simulink model "OverlapSaveFIR_11paths"  (R2024a)
settings: Solver=VariableStepAuto  StartTime=0.0  StopTime=8192  RelTol=1e-3
InitFcn:
  | N=256;
  | h=firpm(128,[0;0.4;0.5;1],[1;1;0;0],[1;50],{20});
  | hc=fft(h,N);
  | h_quant = int16(2^14*hc/max(hc));
  | M=length(h);
values from neighbouring files (symbols this model uses):
  tmp = double(int16(tmp*2^16))/2^16    [test_tap32_fft128.m]
undefined symbols (not defined in the file or in its folder): S, vsva2197, xcvc1902
libraries: aieBasic x44, aieUtilities x11, dspxfrm3 x2, dspsrcs4 x2, vmcUtilities x1
(part 2 of 2)

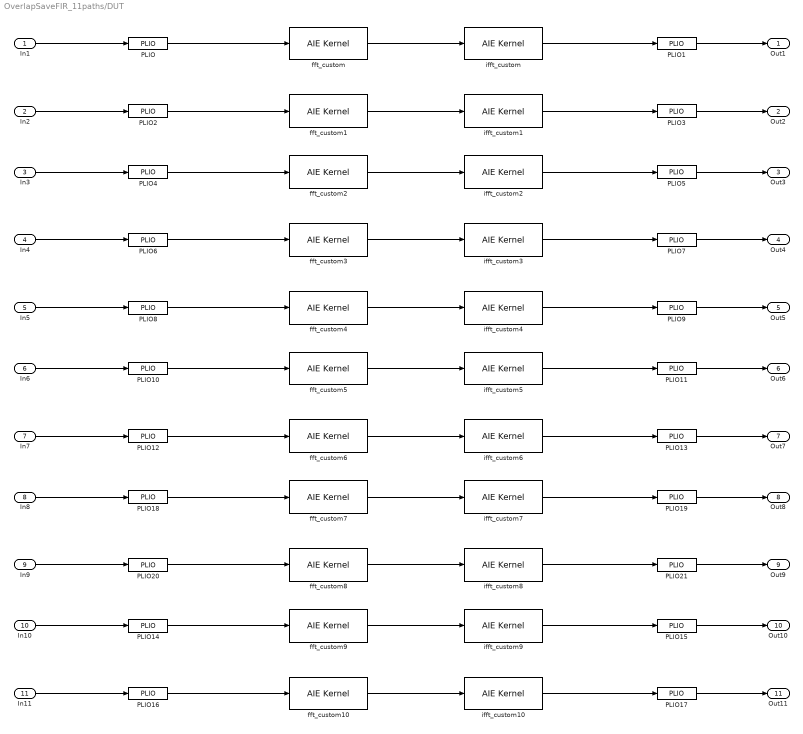
== system OverlapSaveFIR_11paths/DUT ==
  In1 : Inport
  In2 : Inport  Port=2
  In3 : Inport  Port=3
  In4 : Inport  Port=4
  In5 : Inport  Port=5
  In6 : Inport  Port=6
  In7 : Inport  Port=7
  In8 : Inport  Port=8
  In9 : Inport  Port=9
  In10 : Inport  Port=10
  In11 : Inport  Port=11
  PLIO{,1..21} (22 alike) : aieBasic/PLIO  PlioWidth=64  PlioFreqSpec=on  PlioFreq=625  ColLocation=0  channel=0  blockJsonConstraints=[]  deprecateConstraints=0
  fft_custom : aieBasic/AIE Kernel  KernelAllAttrs=s[12;12;9;9;19;14;21;23;21;23;24;21;15;17;12;24;26;26;26;27;28;9;21;23;23;23;24;25;14;19;19;29]@FunctionNameDeclFileNamePortNamesPortTypesPortSerializedTypesPortDirectionsPortWindowSizeEnablesPortWindowMarginEnablesPortBufferSizeEnablesPortBufferMarginEnablesPortSynchronicityEnablesPortSignalSizeEnablesPortBufferSizesPortBufferMarginsFunctionDeclFunctionTemplateSpecKindFunctionTemplateParamNamesFunctionTemplateParamKindsFunctionTemplateParamTypesFunctionTemplateParamValuesFunctionTemplateParamEnablesClassDeclClassTemplateSpecKindClassTemplateParamNamesClassTemplateParamKindsClassTemplateParamTypesClassTemplateParamValuesClassTemplateParamEnablesClassCtorDeclsClassCtorParamNamesClassCtorParamTypesClassCtorParamSerializedTypes[1 1]@C[32 1]@t10@fft_customt33@../../customFFT_casc/fft_custom.hC[2 1]@t5@sig_it5@sig_oC[2 1]@t59@adf::input_buffer< cint32, adf::extents< 256 > > & restrictt32@output_cascade< cacc48, void > *C[2 1]@t71@{Q2{R{Tadf::input_buffer{2{t{Scint32}}{t{Tadf::extents{1{t{}256}}}}}}}}t42@{P{Toutput_cascade{2{t{Scacc48}}{t{Bv}}}}}C[2 1]@t5@inputt6@outputC[2 1]@l1@l0@C[2 1]@l1@l0@C[2 1]@l1@l0@C[2 1]@l0@l0@C[2 1]@l1@l0@C[2 1]@l0@l1@C[2 1]@t3@256nC[2 1]@nnt122@void fft_custom(adf::input_buffer< cint32, adf::extents< 256 > > & restrict sig_i, output_cascade< cacc48, void > * sig_o)t4@nonee[0 1]@e[0 1]@e[0 1]@e[0 1]@e[0 1]@nne[0 1]@e[0 1]@e[0 1]@e[0 1]@e[0 1]@e[0 1]@e[0 1]@e[0 1]@e[0 1]@  PortNames={'sig_i'; 'sig_o'}  PortSerializedTypes={'{Q2{R{Tadf::input_buffer{2{t{Scint32}}{t{Tadf::extents{1{t{}256}}}}}}}}'; '{P{Toutput_cascade{2{t{Scacc48}}{t{Bv}}}}}'}  PortWindowSizes={2.560000000000000000e+02, 0.000000000000000000e+00}  PortWindowMargins={0.000000000000000000e+00, 0.000000000000000000e+00}  PortSynchronicities={'sync', 'auto'}  PortSignalSizes={0.000000000000000000e+00; 2.560000000000000000e+02}  FunctionTemplateSpecKind=none  FunctionTemplateParamNames={}  FunctionTemplateParamKinds={}  FunctionTemplateParamTypes={}  FunctionTemplateParamValues={}  FunctionIndex=1  FunctionTabVisible=on  FunctionTemplateParamsVisible=off  FunctionDeclTypeOptions=C[1 1]@t123@void fft_custom(adf::input_buffer< cint32, adf::extents< 256 > > && restrict sig_i, output_cascade< cacc48, void > * sig_o)  FunctionDecl=void fft_custom(adf::input_buffer< cint32, adf::extents< 256 > > && restrict sig_i, output_cascade< cacc48, void > * sig_o)  FunctionTemplateParams={}  FunctionTemplateParamsEnables={}  PortAttrs={ 'input', 'sig_i', 'adf::input_buffer< cint32, adf::extents< 256 > > & restrict', '256', '0', 'sync', ''; 'output', 'sig_o', 'output_cascade< cacc48, void > *', '', '', '', '256' }  PortAttrsEnables={'off', 'off', 'off', 'off', 'off', 'off', 'off';'off', 'off', 'off', 'off', 'off', 'off', 'on'}  SampleTime=-1  KernelHeaderFile=customFFT_casc/fft_custom.h  KernelFunction=fft_custom  KernelInitFunction=fft_custom_init  KernelSourceFile=customFFT_casc/fft_custom.cpp  KernelSearchPaths={'./customFFT_casc'}  PreProcOptions={}  blockJsonConstraints="{\"type\":\"constraint\",\"constraintType\":\"stackSize\",\"sid\":\"5803\",\"lhs\":{\"type\":\"stackSize\",\"args\":{\"type\":\"kernel\",\"name\":\"OverlapSaveFIR_11paths/custom_11copies/fft_custom\",\"sid\":\"5803\"}},\"rhs\":{\"type\":\"value\",\"args\":{\"type\":\"evaluable\",\"expr\":\"3200\",\"value\":3200}},\"equality\":true}"
  fft_custom1 : aieBasic/AIE Kernel  KernelAllAttrs=s[12;12;9;9;19;14;21;23;21;23;24;21;15;17;12;24;26;26;26;27;28;9;21;23;23;23;24;25;14;19;19;29]@FunctionNameDeclFileNamePortNamesPortTypesPortSerializedTypesPortDirectionsPortWindowSizeEnablesPortWindowMarginEnablesPortBufferSizeEnablesPortBufferMarginEnablesPortSynchronicityEnablesPortSignalSizeEnablesPortBufferSizesPortBufferMarginsFunctionDeclFunctionTemplateSpecKindFunctionTemplateParamNamesFunctionTemplateParamKindsFunctionTemplateParamTypesFunctionTemplateParamValuesFunctionTemplateParamEnablesClassDeclClassTemplateSpecKindClassTemplateParamNamesClassTemplateParamKindsClassTemplateParamTypesClassTemplateParamValuesClassTemplateParamEnablesClassCtorDeclsClassCtorParamNamesClassCtorParamTypesClassCtorParamSerializedTypes[1 1]@C[32 1]@t10@fft_customt33@../../customFFT_casc/fft_custom.hC[2 1]@t5@sig_it5@sig_oC[2 1]@t59@adf::input_buffer< cint32, adf::extents< 256 > > & restrictt32@output_cascade< cacc48, void > *C[2 1]@t71@{Q2{R{Tadf::input_buffer{2{t{Scint32}}{t{Tadf::extents{1{t{}256}}}}}}}}t42@{P{Toutput_cascade{2{t{Scacc48}}{t{Bv}}}}}C[2 1]@t5@inputt6@outputC[2 1]@l1@l0@C[2 1]@l1@l0@C[2 1]@l1@l0@C[2 1]@l0@l0@C[2 1]@l1@l0@C[2 1]@l0@l1@C[2 1]@t3@256nC[2 1]@nnt122@void fft_custom(adf::input_buffer< cint32, adf::extents< 256 > > & restrict sig_i, output_cascade< cacc48, void > * sig_o)t4@nonee[0 1]@e[0 1]@e[0 1]@e[0 1]@e[0 1]@nne[0 1]@e[0 1]@e[0 1]@e[0 1]@e[0 1]@e[0 1]@e[0 1]@e[0 1]@e[0 1]@  PortNames={'sig_i'; 'sig_o'}  PortSerializedTypes={'{Q2{R{Tadf::input_buffer{2{t{Scint32}}{t{Tadf::extents{1{t{}256}}}}}}}}'; '{P{Toutput_cascade{2{t{Scacc48}}{t{Bv}}}}}'}  PortWindowSizes={2.560000000000000000e+02, 0.000000000000000000e+00}  PortWindowMargins={0.000000000000000000e+00, 0.000000000000000000e+00}  PortSynchronicities={'sync', 'auto'}  PortSignalSizes={0.000000000000000000e+00; 2.560000000000000000e+02}  FunctionTemplateSpecKind=none  FunctionTemplateParamNames={}  FunctionTemplateParamKinds={}  FunctionTemplateParamTypes={}  FunctionTemplateParamValues={}  FunctionIndex=1  FunctionTabVisible=on  FunctionTemplateParamsVisible=off  FunctionDeclTypeOptions=C[1 1]@t123@void fft_custom(adf::input_buffer< cint32, adf::extents< 256 > > && restrict sig_i, output_cascade< cacc48, void > * sig_o)  FunctionDecl=void fft_custom(adf::input_buffer< cint32, adf::extents< 256 > > && restrict sig_i, output_cascade< cacc48, void > * sig_o)  FunctionTemplateParams={}  FunctionTemplateParamsEnables={}  PortAttrs={ 'input', 'sig_i', 'adf::input_buffer< cint32, adf::extents< 256 > > & restrict', '256', '0', 'sync', ''; 'output', 'sig_o', 'output_cascade< cacc48, void > *', '', '', '', '256' }  PortAttrsEnables={'off', 'off', 'off', 'off', 'off', 'off', 'off';'off', 'off', 'off', 'off', 'off', 'off', 'on'}  SampleTime=-1  KernelHeaderFile=customFFT_casc/fft_custom.h  KernelFunction=fft_custom  KernelInitFunction=fft_custom_init  KernelSourceFile=customFFT_casc/fft_custom.cpp  KernelSearchPaths={'./customFFT_casc'}  PreProcOptions={}  blockJsonConstraints="{\"type\":\"constraint\",\"constraintType\":\"stackSize\",\"sid\":\"5804\",\"lhs\":{\"type\":\"stackSize\",\"args\":{\"type\":\"kernel\",\"name\":\"OverlapSaveFIR_11paths/custom_11copies/fft_custom1\",\"sid\":\"5804\"}},\"rhs\":{\"type\":\"value\",\"args\":{\"type\":\"evaluable\",\"expr\":\"3200\",\"value\":3200}},\"equality\":true}"
  fft_custom10 : aieBasic/AIE Kernel  KernelAllAttrs=s[12;12;9;9;19;14;21;23;21;23;24;21;15;17;12;24;26;26;26;27;28;9;21;23;23;23;24;25;14;19;19;29]@FunctionNameDeclFileNamePortNamesPortTypesPortSerializedTypesPortDirectionsPortWindowSizeEnablesPortWindowMarginEnablesPortBufferSizeEnablesPortBufferMarginEnablesPortSynchronicityEnablesPortSignalSizeEnablesPortBufferSizesPortBufferMarginsFunctionDeclFunctionTemplateSpecKindFunctionTemplateParamNamesFunctionTemplateParamKindsFunctionTemplateParamTypesFunctionTemplateParamValuesFunctionTemplateParamEnablesClassDeclClassTemplateSpecKindClassTemplateParamNamesClassTemplateParamKindsClassTemplateParamTypesClassTemplateParamValuesClassTemplateParamEnablesClassCtorDeclsClassCtorParamNamesClassCtorParamTypesClassCtorParamSerializedTypes[1 1]@C[32 1]@t10@fft_customt33@../../customFFT_casc/fft_custom.hC[2 1]@t5@sig_it5@sig_oC[2 1]@t59@adf::input_buffer< cint32, adf::extents< 256 > > & restrictt32@output_cascade< cacc48, void > *C[2 1]@t71@{Q2{R{Tadf::input_buffer{2{t{Scint32}}{t{Tadf::extents{1{t{}256}}}}}}}}t42@{P{Toutput_cascade{2{t{Scacc48}}{t{Bv}}}}}C[2 1]@t5@inputt6@outputC[2 1]@l1@l0@C[2 1]@l1@l0@C[2 1]@l1@l0@C[2 1]@l0@l0@C[2 1]@l1@l0@C[2 1]@l0@l1@C[2 1]@t3@256nC[2 1]@nnt122@void fft_custom(adf::input_buffer< cint32, adf::extents< 256 > > & restrict sig_i, output_cascade< cacc48, void > * sig_o)t4@nonee[0 1]@e[0 1]@e[0 1]@e[0 1]@e[0 1]@nne[0 1]@e[0 1]@e[0 1]@e[0 1]@e[0 1]@e[0 1]@e[0 1]@e[0 1]@e[0 1]@  PortNames={'sig_i'; 'sig_o'}  PortSerializedTypes={'{Q2{R{Tadf::input_buffer{2{t{Scint32}}{t{Tadf::extents{1{t{}256}}}}}}}}'; '{P{Toutput_cascade{2{t{Scacc48}}{t{Bv}}}}}'}  PortWindowSizes={2.560000000000000000e+02, 0.000000000000000000e+00}  PortWindowMargins={0.000000000000000000e+00, 0.000000000000000000e+00}  PortSynchronicities={'sync', 'auto'}  PortSignalSizes={0.000000000000000000e+00; 2.560000000000000000e+02}  FunctionTemplateSpecKind=none  FunctionTemplateParamNames={}  FunctionTemplateParamKinds={}  FunctionTemplateParamTypes={}  FunctionTemplateParamValues={}  FunctionIndex=1  FunctionTabVisible=on  FunctionTemplateParamsVisible=off  FunctionDeclTypeOptions=C[1 1]@t123@void fft_custom(adf::input_buffer< cint32, adf::extents< 256 > > && restrict sig_i, output_cascade< cacc48, void > * sig_o)  FunctionDecl=void fft_custom(adf::input_buffer< cint32, adf::extents< 256 > > && restrict sig_i, output_cascade< cacc48, void > * sig_o)  FunctionTemplateParams={}  FunctionTemplateParamsEnables={}  PortAttrs={ 'input', 'sig_i', 'adf::input_buffer< cint32, adf::extents< 256 > > & restrict', '256', '0', 'sync', ''; 'output', 'sig_o', 'output_cascade< cacc48, void > *', '', '', '', '256' }  PortAttrsEnables={'off', 'off', 'off', 'off', 'off', 'off', 'off';'off', 'off', 'off', 'off', 'off', 'off', 'on'}  SampleTime=-1  KernelHeaderFile=customFFT_casc/fft_custom.h  KernelFunction=fft_custom  KernelInitFunction=fft_custom_init  KernelSourceFile=customFFT_casc/fft_custom.cpp  KernelSearchPaths={'./customFFT_casc'}  PreProcOptions={}  blockJsonConstraints="{\"type\":\"constraint\",\"constraintType\":\"stackSize\",\"sid\":\"5805\",\"lhs\":{\"type\":\"stackSize\",\"args\":{\"type\":\"kernel\",\"name\":\"OverlapSaveFIR_11paths/custom_11copies/fft_custom10\",\"sid\":\"5805\"}},\"rhs\":{\"type\":\"value\",\"args\":{\"type\":\"evaluable\",\"expr\":\"3200\",\"value\":3200}},\"equality\":true}"
  fft_custom2 : aieBasic/AIE Kernel  KernelAllAttrs=s[12;12;9;9;19;14;21;23;21;23;24;21;15;17;12;24;26;26;26;27;28;9;21;23;23;23;24;25;14;19;19;29]@FunctionNameDeclFileNamePortNamesPortTypesPortSerializedTypesPortDirectionsPortWindowSizeEnablesPortWindowMarginEnablesPortBufferSizeEnablesPortBufferMarginEnablesPortSynchronicityEnablesPortSignalSizeEnablesPortBufferSizesPortBufferMarginsFunctionDeclFunctionTemplateSpecKindFunctionTemplateParamNamesFunctionTemplateParamKindsFunctionTemplateParamTypesFunctionTemplateParamValuesFunctionTemplateParamEnablesClassDeclClassTemplateSpecKindClassTemplateParamNamesClassTemplateParamKindsClassTemplateParamTypesClassTemplateParamValuesClassTemplateParamEnablesClassCtorDeclsClassCtorParamNamesClassCtorParamTypesClassCtorParamSerializedTypes[1 1]@C[32 1]@t10@fft_customt33@../../customFFT_casc/fft_custom.hC[2 1]@t5@sig_it5@sig_oC[2 1]@t59@adf::input_buffer< cint32, adf::extents< 256 > > & restrictt32@output_cascade< cacc48, void > *C[2 1]@t71@{Q2{R{Tadf::input_buffer{2{t{Scint32}}{t{Tadf::extents{1{t{}256}}}}}}}}t42@{P{Toutput_cascade{2{t{Scacc48}}{t{Bv}}}}}C[2 1]@t5@inputt6@outputC[2 1]@l1@l0@C[2 1]@l1@l0@C[2 1]@l1@l0@C[2 1]@l0@l0@C[2 1]@l1@l0@C[2 1]@l0@l1@C[2 1]@t3@256nC[2 1]@nnt122@void fft_custom(adf::input_buffer< cint32, adf::extents< 256 > > & restrict sig_i, output_cascade< cacc48, void > * sig_o)t4@nonee[0 1]@e[0 1]@e[0 1]@e[0 1]@e[0 1]@nne[0 1]@e[0 1]@e[0 1]@e[0 1]@e[0 1]@e[0 1]@e[0 1]@e[0 1]@e[0 1]@  PortNames={'sig_i'; 'sig_o'}  PortSerializedTypes={'{Q2{R{Tadf::input_buffer{2{t{Scint32}}{t{Tadf::extents{1{t{}256}}}}}}}}'; '{P{Toutput_cascade{2{t{Scacc48}}{t{Bv}}}}}'}  PortWindowSizes={2.560000000000000000e+02, 0.000000000000000000e+00}  PortWindowMargins={0.000000000000000000e+00, 0.000000000000000000e+00}  PortSynchronicities={'sync', 'auto'}  PortSignalSizes={0.000000000000000000e+00; 2.560000000000000000e+02}  FunctionTemplateSpecKind=none  FunctionTemplateParamNames={}  FunctionTemplateParamKinds={}  FunctionTemplateParamTypes={}  FunctionTemplateParamValues={}  FunctionIndex=1  FunctionTabVisible=on  FunctionTemplateParamsVisible=off  FunctionDeclTypeOptions=C[1 1]@t123@void fft_custom(adf::input_buffer< cint32, adf::extents< 256 > > && restrict sig_i, output_cascade< cacc48, void > * sig_o)  FunctionDecl=void fft_custom(adf::input_buffer< cint32, adf::extents< 256 > > && restrict sig_i, output_cascade< cacc48, void > * sig_o)  FunctionTemplateParams={}  FunctionTemplateParamsEnables={}  PortAttrs={ 'input', 'sig_i', 'adf::input_buffer< cint32, adf::extents< 256 > > & restrict', '256', '0', 'sync', ''; 'output', 'sig_o', 'output_cascade< cacc48, void > *', '', '', '', '256' }  PortAttrsEnables={'off', 'off', 'off', 'off', 'off', 'off', 'off';'off', 'off', 'off', 'off', 'off', 'off', 'on'}  SampleTime=-1  KernelHeaderFile=customFFT_casc/fft_custom.h  KernelFunction=fft_custom  KernelInitFunction=fft_custom_init  KernelSourceFile=customFFT_casc/fft_custom.cpp  KernelSearchPaths={'./customFFT_casc'}  PreProcOptions={}  blockJsonConstraints="{\"type\":\"constraint\",\"constraintType\":\"stackSize\",\"sid\":\"5806\",\"lhs\":{\"type\":\"stackSize\",\"args\":{\"type\":\"kernel\",\"name\":\"OverlapSaveFIR_11paths/custom_11copies/fft_custom2\",\"sid\":\"5806\"}},\"rhs\":{\"type\":\"value\",\"args\":{\"type\":\"evaluable\",\"expr\":\"3200\",\"value\":3200}},\"equality\":true}"
  fft_custom3 : aieBasic/AIE Kernel  KernelAllAttrs=s[12;12;9;9;19;14;21;23;21;23;24;21;15;17;12;24;26;26;26;27;28;9;21;23;23;23;24;25;14;19;19;29]@FunctionNameDeclFileNamePortNamesPortTypesPortSerializedTypesPortDirectionsPortWindowSizeEnablesPortWindowMarginEnablesPortBufferSizeEnablesPortBufferMarginEnablesPortSynchronicityEnablesPortSignalSizeEnablesPortBufferSizesPortBufferMarginsFunctionDeclFunctionTemplateSpecKindFunctionTemplateParamNamesFunctionTemplateParamKindsFunctionTemplateParamTypesFunctionTemplateParamValuesFunctionTemplateParamEnablesClassDeclClassTemplateSpecKindClassTemplateParamNamesClassTemplateParamKindsClassTemplateParamTypesClassTemplateParamValuesClassTemplateParamEnablesClassCtorDeclsClassCtorParamNamesClassCtorParamTypesClassCtorParamSerializedTypes[1 1]@C[32 1]@t10@fft_customt33@../../customFFT_casc/fft_custom.hC[2 1]@t5@sig_it5@sig_oC[2 1]@t59@adf::input_buffer< cint32, adf::extents< 256 > > & restrictt32@output_cascade< cacc48, void > *C[2 1]@t71@{Q2{R{Tadf::input_buffer{2{t{Scint32}}{t{Tadf::extents{1{t{}256}}}}}}}}t42@{P{Toutput_cascade{2{t{Scacc48}}{t{Bv}}}}}C[2 1]@t5@inputt6@outputC[2 1]@l1@l0@C[2 1]@l1@l0@C[2 1]@l1@l0@C[2 1]@l0@l0@C[2 1]@l1@l0@C[2 1]@l0@l1@C[2 1]@t3@256nC[2 1]@nnt122@void fft_custom(adf::input_buffer< cint32, adf::extents< 256 > > & restrict sig_i, output_cascade< cacc48, void > * sig_o)t4@nonee[0 1]@e[0 1]@e[0 1]@e[0 1]@e[0 1]@nne[0 1]@e[0 1]@e[0 1]@e[0 1]@e[0 1]@e[0 1]@e[0 1]@e[0 1]@e[0 1]@  PortNames={'sig_i'; 'sig_o'}  PortSerializedTypes={'{Q2{R{Tadf::input_buffer{2{t{Scint32}}{t{Tadf::extents{1{t{}256}}}}}}}}'; '{P{Toutput_cascade{2{t{Scacc48}}{t{Bv}}}}}'}  PortWindowSizes={2.560000000000000000e+02, 0.000000000000000000e+00}  PortWindowMargins={0.000000000000000000e+00, 0.000000000000000000e+00}  PortSynchronicities={'sync', 'auto'}  PortSignalSizes={0.000000000000000000e+00; 2.560000000000000000e+02}  FunctionTemplateSpecKind=none  FunctionTemplateParamNames={}  FunctionTemplateParamKinds={}  FunctionTemplateParamTypes={}  FunctionTemplateParamValues={}  FunctionIndex=1  FunctionTabVisible=on  FunctionTemplateParamsVisible=off  FunctionDeclTypeOptions=C[1 1]@t123@void fft_custom(adf::input_buffer< cint32, adf::extents< 256 > > && restrict sig_i, output_cascade< cacc48, void > * sig_o)  FunctionDecl=void fft_custom(adf::input_buffer< cint32, adf::extents< 256 > > && restrict sig_i, output_cascade< cacc48, void > * sig_o)  FunctionTemplateParams={}  FunctionTemplateParamsEnables={}  PortAttrs={ 'input', 'sig_i', 'adf::input_buffer< cint32, adf::extents< 256 > > & restrict', '256', '0', 'sync', ''; 'output', 'sig_o', 'output_cascade< cacc48, void > *', '', '', '', '256' }  PortAttrsEnables={'off', 'off', 'off', 'off', 'off', 'off', 'off';'off', 'off', 'off', 'off', 'off', 'off', 'on'}  SampleTime=-1  KernelHeaderFile=customFFT_casc/fft_custom.h  KernelFunction=fft_custom  KernelInitFunction=fft_custom_init  KernelSourceFile=customFFT_casc/fft_custom.cpp  KernelSearchPaths={'./customFFT_casc'}  PreProcOptions={}  blockJsonConstraints="{\"type\":\"constraint\",\"constraintType\":\"stackSize\",\"sid\":\"5807\",\"lhs\":{\"type\":\"stackSize\",\"args\":{\"type\":\"kernel\",\"name\":\"OverlapSaveFIR_11paths/custom_11copies/fft_custom3\",\"sid\":\"5807\"}},\"rhs\":{\"type\":\"value\",\"args\":{\"type\":\"evaluable\",\"expr\":\"3200\",\"value\":3200}},\"equality\":true}"
  fft_custom4 : aieBasic/AIE Kernel  KernelAllAttrs=s[12;12;9;9;19;14;21;23;21;23;24;21;15;17;12;24;26;26;26;27;28;9;21;23;23;23;24;25;14;19;19;29]@FunctionNameDeclFileNamePortNamesPortTypesPortSerializedTypesPortDirectionsPortWindowSizeEnablesPortWindowMarginEnablesPortBufferSizeEnablesPortBufferMarginEnablesPortSynchronicityEnablesPortSignalSizeEnablesPortBufferSizesPortBufferMarginsFunctionDeclFunctionTemplateSpecKindFunctionTemplateParamNamesFunctionTemplateParamKindsFunctionTemplateParamTypesFunctionTemplateParamValuesFunctionTemplateParamEnablesClassDeclClassTemplateSpecKindClassTemplateParamNamesClassTemplateParamKindsClassTemplateParamTypesClassTemplateParamValuesClassTemplateParamEnablesClassCtorDeclsClassCtorParamNamesClassCtorParamTypesClassCtorParamSerializedTypes[1 1]@C[32 1]@t10@fft_customt33@../../customFFT_casc/fft_custom.hC[2 1]@t5@sig_it5@sig_oC[2 1]@t59@adf::input_buffer< cint32, adf::extents< 256 > > & restrictt32@output_cascade< cacc48, void > *C[2 1]@t71@{Q2{R{Tadf::input_buffer{2{t{Scint32}}{t{Tadf::extents{1{t{}256}}}}}}}}t42@{P{Toutput_cascade{2{t{Scacc48}}{t{Bv}}}}}C[2 1]@t5@inputt6@outputC[2 1]@l1@l0@C[2 1]@l1@l0@C[2 1]@l1@l0@C[2 1]@l0@l0@C[2 1]@l1@l0@C[2 1]@l0@l1@C[2 1]@t3@256nC[2 1]@nnt122@void fft_custom(adf::input_buffer< cint32, adf::extents< 256 > > & restrict sig_i, output_cascade< cacc48, void > * sig_o)t4@nonee[0 1]@e[0 1]@e[0 1]@e[0 1]@e[0 1]@nne[0 1]@e[0 1]@e[0 1]@e[0 1]@e[0 1]@e[0 1]@e[0 1]@e[0 1]@e[0 1]@  PortNames={'sig_i'; 'sig_o'}  PortSerializedTypes={'{Q2{R{Tadf::input_buffer{2{t{Scint32}}{t{Tadf::extents{1{t{}256}}}}}}}}'; '{P{Toutput_cascade{2{t{Scacc48}}{t{Bv}}}}}'}  PortWindowSizes={2.560000000000000000e+02, 0.000000000000000000e+00}  PortWindowMargins={0.000000000000000000e+00, 0.000000000000000000e+00}  PortSynchronicities={'sync', 'auto'}  PortSignalSizes={0.000000000000000000e+00; 2.560000000000000000e+02}  FunctionTemplateSpecKind=none  FunctionTemplateParamNames={}  FunctionTemplateParamKinds={}  FunctionTemplateParamTypes={}  FunctionTemplateParamValues={}  FunctionIndex=1  FunctionTabVisible=on  FunctionTemplateParamsVisible=off  FunctionDeclTypeOptions=C[1 1]@t123@void fft_custom(adf::input_buffer< cint32, adf::extents< 256 > > && restrict sig_i, output_cascade< cacc48, void > * sig_o)  FunctionDecl=void fft_custom(adf::input_buffer< cint32, adf::extents< 256 > > && restrict sig_i, output_cascade< cacc48, void > * sig_o)  FunctionTemplateParams={}  FunctionTemplateParamsEnables={}  PortAttrs={ 'input', 'sig_i', 'adf::input_buffer< cint32, adf::extents< 256 > > & restrict', '256', '0', 'sync', ''; 'output', 'sig_o', 'output_cascade< cacc48, void > *', '', '', '', '256' }  PortAttrsEnables={'off', 'off', 'off', 'off', 'off', 'off', 'off';'off', 'off', 'off', 'off', 'off', 'off', 'on'}  SampleTime=-1  KernelHeaderFile=customFFT_casc/fft_custom.h  KernelFunction=fft_custom  KernelInitFunction=fft_custom_init  KernelSourceFile=customFFT_casc/fft_custom.cpp  KernelSearchPaths={'./customFFT_casc'}  PreProcOptions={}  blockJsonConstraints="{\"type\":\"constraint\",\"constraintType\":\"stackSize\",\"sid\":\"5808\",\"lhs\":{\"type\":\"stackSize\",\"args\":{\"type\":\"kernel\",\"name\":\"OverlapSaveFIR_11paths/custom_11copies/fft_custom4\",\"sid\":\"5808\"}},\"rhs\":{\"type\":\"value\",\"args\":{\"type\":\"evaluable\",\"expr\":\"3200\",\"value\":3200}},\"equality\":true}"
  fft_custom5 : aieBasic/AIE Kernel  KernelAllAttrs=s[12;12;9;9;19;14;21;23;21;23;24;21;15;17;12;24;26;26;26;27;28;9;21;23;23;23;24;25;14;19;19;29]@FunctionNameDeclFileNamePortNamesPortTypesPortSerializedTypesPortDirectionsPortWindowSizeEnablesPortWindowMarginEnablesPortBufferSizeEnablesPortBufferMarginEnablesPortSynchronicityEnablesPortSignalSizeEnablesPortBufferSizesPortBufferMarginsFunctionDeclFunctionTemplateSpecKindFunctionTemplateParamNamesFunctionTemplateParamKindsFunctionTemplateParamTypesFunctionTemplateParamValuesFunctionTemplateParamEnablesClassDeclClassTemplateSpecKindClassTemplateParamNamesClassTemplateParamKindsClassTemplateParamTypesClassTemplateParamValuesClassTemplateParamEnablesClassCtorDeclsClassCtorParamNamesClassCtorParamTypesClassCtorParamSerializedTypes[1 1]@C[32 1]@t10@fft_customt33@../../customFFT_casc/fft_custom.hC[2 1]@t5@sig_it5@sig_oC[2 1]@t59@adf::input_buffer< cint32, adf::extents< 256 > > & restrictt32@output_cascade< cacc48, void > *C[2 1]@t71@{Q2{R{Tadf::input_buffer{2{t{Scint32}}{t{Tadf::extents{1{t{}256}}}}}}}}t42@{P{Toutput_cascade{2{t{Scacc48}}{t{Bv}}}}}C[2 1]@t5@inputt6@outputC[2 1]@l1@l0@C[2 1]@l1@l0@C[2 1]@l1@l0@C[2 1]@l0@l0@C[2 1]@l1@l0@C[2 1]@l0@l1@C[2 1]@t3@256nC[2 1]@nnt122@void fft_custom(adf::input_buffer< cint32, adf::extents< 256 > > & restrict sig_i, output_cascade< cacc48, void > * sig_o)t4@nonee[0 1]@e[0 1]@e[0 1]@e[0 1]@e[0 1]@nne[0 1]@e[0 1]@e[0 1]@e[0 1]@e[0 1]@e[0 1]@e[0 1]@e[0 1]@e[0 1]@  PortNames={'sig_i'; 'sig_o'}  PortSerializedTypes={'{Q2{R{Tadf::input_buffer{2{t{Scint32}}{t{Tadf::extents{1{t{}256}}}}}}}}'; '{P{Toutput_cascade{2{t{Scacc48}}{t{Bv}}}}}'}  PortWindowSizes={2.560000000000000000e+02, 0.000000000000000000e+00}  PortWindowMargins={0.000000000000000000e+00, 0.000000000000000000e+00}  PortSynchronicities={'sync', 'auto'}  PortSignalSizes={0.000000000000000000e+00; 2.560000000000000000e+02}  FunctionTemplateSpecKind=none  FunctionTemplateParamNames={}  FunctionTemplateParamKinds={}  FunctionTemplateParamTypes={}  FunctionTemplateParamValues={}  FunctionIndex=1  FunctionTabVisible=on  FunctionTemplateParamsVisible=off  FunctionDeclTypeOptions=C[1 1]@t123@void fft_custom(adf::input_buffer< cint32, adf::extents< 256 > > && restrict sig_i, output_cascade< cacc48, void > * sig_o)  FunctionDecl=void fft_custom(adf::input_buffer< cint32, adf::extents< 256 > > && restrict sig_i, output_cascade< cacc48, void > * sig_o)  FunctionTemplateParams={}  FunctionTemplateParamsEnables={}  PortAttrs={ 'input', 'sig_i', 'adf::input_buffer< cint32, adf::extents< 256 > > & restrict', '256', '0', 'sync', ''; 'output', 'sig_o', 'output_cascade< cacc48, void > *', '', '', '', '256' }  PortAttrsEnables={'off', 'off', 'off', 'off', 'off', 'off', 'off';'off', 'off', 'off', 'off', 'off', 'off', 'on'}  SampleTime=-1  KernelHeaderFile=customFFT_casc/fft_custom.h  KernelFunction=fft_custom  KernelInitFunction=fft_custom_init  KernelSourceFile=customFFT_casc/fft_custom.cpp  KernelSearchPaths={'./customFFT_casc'}  PreProcOptions={}  blockJsonConstraints="{\"type\":\"constraint\",\"constraintType\":\"stackSize\",\"sid\":\"5809\",\"lhs\":{\"type\":\"stackSize\",\"args\":{\"type\":\"kernel\",\"name\":\"OverlapSaveFIR_11paths/custom_11copies/fft_custom5\",\"sid\":\"5809\"}},\"rhs\":{\"type\":\"value\",\"args\":{\"type\":\"evaluable\",\"expr\":\"3200\",\"value\":3200}},\"equality\":true}"
  fft_custom6 : aieBasic/AIE Kernel  KernelAllAttrs=s[12;12;9;9;19;14;21;23;21;23;24;21;15;17;12;24;26;26;26;27;28;9;21;23;23;23;24;25;14;19;19;29]@FunctionNameDeclFileNamePortNamesPortTypesPortSerializedTypesPortDirectionsPortWindowSizeEnablesPortWindowMarginEnablesPortBufferSizeEnablesPortBufferMarginEnablesPortSynchronicityEnablesPortSignalSizeEnablesPortBufferSizesPortBufferMarginsFunctionDeclFunctionTemplateSpecKindFunctionTemplateParamNamesFunctionTemplateParamKindsFunctionTemplateParamTypesFunctionTemplateParamValuesFunctionTemplateParamEnablesClassDeclClassTemplateSpecKindClassTemplateParamNamesClassTemplateParamKindsClassTemplateParamTypesClassTemplateParamValuesClassTemplateParamEnablesClassCtorDeclsClassCtorParamNamesClassCtorParamTypesClassCtorParamSerializedTypes[1 1]@C[32 1]@t10@fft_customt33@../../customFFT_casc/fft_custom.hC[2 1]@t5@sig_it5@sig_oC[2 1]@t59@adf::input_buffer< cint32, adf::extents< 256 > > & restrictt32@output_cascade< cacc48, void > *C[2 1]@t71@{Q2{R{Tadf::input_buffer{2{t{Scint32}}{t{Tadf::extents{1{t{}256}}}}}}}}t42@{P{Toutput_cascade{2{t{Scacc48}}{t{Bv}}}}}C[2 1]@t5@inputt6@outputC[2 1]@l1@l0@C[2 1]@l1@l0@C[2 1]@l1@l0@C[2 1]@l0@l0@C[2 1]@l1@l0@C[2 1]@l0@l1@C[2 1]@t3@256nC[2 1]@nnt122@void fft_custom(adf::input_buffer< cint32, adf::extents< 256 > > & restrict sig_i, output_cascade< cacc48, void > * sig_o)t4@nonee[0 1]@e[0 1]@e[0 1]@e[0 1]@e[0 1]@nne[0 1]@e[0 1]@e[0 1]@e[0 1]@e[0 1]@e[0 1]@e[0 1]@e[0 1]@e[0 1]@  PortNames={'sig_i'; 'sig_o'}  PortSerializedTypes={'{Q2{R{Tadf::input_buffer{2{t{Scint32}}{t{Tadf::extents{1{t{}256}}}}}}}}'; '{P{Toutput_cascade{2{t{Scacc48}}{t{Bv}}}}}'}  PortWindowSizes={2.560000000000000000e+02, 0.000000000000000000e+00}  PortWindowMargins={0.000000000000000000e+00, 0.000000000000000000e+00}  PortSynchronicities={'sync', 'auto'}  PortSignalSizes={0.000000000000000000e+00; 2.560000000000000000e+02}  FunctionTemplateSpecKind=none  FunctionTemplateParamNames={}  FunctionTemplateParamKinds={}  FunctionTemplateParamTypes={}  FunctionTemplateParamValues={}  FunctionIndex=1  FunctionTabVisible=on  FunctionTemplateParamsVisible=off  FunctionDeclTypeOptions=C[1 1]@t123@void fft_custom(adf::input_buffer< cint32, adf::extents< 256 > > && restrict sig_i, output_cascade< cacc48, void > * sig_o)  FunctionDecl=void fft_custom(adf::input_buffer< cint32, adf::extents< 256 > > && restrict sig_i, output_cascade< cacc48, void > * sig_o)  FunctionTemplateParams={}  FunctionTemplateParamsEnables={}  PortAttrs={ 'input', 'sig_i', 'adf::input_buffer< cint32, adf::extents< 256 > > & restrict', '256', '0', 'sync', ''; 'output', 'sig_o', 'output_cascade< cacc48, void > *', '', '', '', '256' }  PortAttrsEnables={'off', 'off', 'off', 'off', 'off', 'off', 'off';'off', 'off', 'off', 'off', 'off', 'off', 'on'}  SampleTime=-1  KernelHeaderFile=customFFT_casc/fft_custom.h  KernelFunction=fft_custom  KernelInitFunction=fft_custom_init  KernelSourceFile=customFFT_casc/fft_custom.cpp  KernelSearchPaths={'./customFFT_casc'}  PreProcOptions={}  blockJsonConstraints="{\"type\":\"constraint\",\"constraintType\":\"stackSize\",\"sid\":\"5810\",\"lhs\":{\"type\":\"stackSize\",\"args\":{\"type\":\"kernel\",\"name\":\"OverlapSaveFIR_11paths/custom_11copies/fft_custom6\",\"sid\":\"5810\"}},\"rhs\":{\"type\":\"value\",\"args\":{\"type\":\"evaluable\",\"expr\":\"3200\",\"value\":3200}},\"equality\":true}"
  fft_custom7 : aieBasic/AIE Kernel  KernelAllAttrs=s[12;12;9;9;19;14;21;23;21;23;24;21;15;17;12;24;26;26;26;27;28;9;21;23;23;23;24;25;14;19;19;29]@FunctionNameDeclFileNamePortNamesPortTypesPortSerializedTypesPortDirectionsPortWindowSizeEnablesPortWindowMarginEnablesPortBufferSizeEnablesPortBufferMarginEnablesPortSynchronicityEnablesPortSignalSizeEnablesPortBufferSizesPortBufferMarginsFunctionDeclFunctionTemplateSpecKindFunctionTemplateParamNamesFunctionTemplateParamKindsFunctionTemplateParamTypesFunctionTemplateParamValuesFunctionTemplateParamEnablesClassDeclClassTemplateSpecKindClassTemplateParamNamesClassTemplateParamKindsClassTemplateParamTypesClassTemplateParamValuesClassTemplateParamEnablesClassCtorDeclsClassCtorParamNamesClassCtorParamTypesClassCtorParamSerializedTypes[1 1]@C[32 1]@t10@fft_customt33@../../customFFT_casc/fft_custom.hC[2 1]@t5@sig_it5@sig_oC[2 1]@t59@adf::input_buffer< cint32, adf::extents< 256 > > & restrictt32@output_cascade< cacc48, void > *C[2 1]@t71@{Q2{R{Tadf::input_buffer{2{t{Scint32}}{t{Tadf::extents{1{t{}256}}}}}}}}t42@{P{Toutput_cascade{2{t{Scacc48}}{t{Bv}}}}}C[2 1]@t5@inputt6@outputC[2 1]@l1@l0@C[2 1]@l1@l0@C[2 1]@l1@l0@C[2 1]@l0@l0@C[2 1]@l1@l0@C[2 1]@l0@l1@C[2 1]@t3@256nC[2 1]@nnt122@void fft_custom(adf::input_buffer< cint32, adf::extents< 256 > > & restrict sig_i, output_cascade< cacc48, void > * sig_o)t4@nonee[0 1]@e[0 1]@e[0 1]@e[0 1]@e[0 1]@nne[0 1]@e[0 1]@e[0 1]@e[0 1]@e[0 1]@e[0 1]@e[0 1]@e[0 1]@e[0 1]@  PortNames={'sig_i'; 'sig_o'}  PortSerializedTypes={'{Q2{R{Tadf::input_buffer{2{t{Scint32}}{t{Tadf::extents{1{t{}256}}}}}}}}'; '{P{Toutput_cascade{2{t{Scacc48}}{t{Bv}}}}}'}  PortWindowSizes={2.560000000000000000e+02, 0.000000000000000000e+00}  PortWindowMargins={0.000000000000000000e+00, 0.000000000000000000e+00}  PortSynchronicities={'sync', 'auto'}  PortSignalSizes={0.000000000000000000e+00; 2.560000000000000000e+02}  FunctionTemplateSpecKind=none  FunctionTemplateParamNames={}  FunctionTemplateParamKinds={}  FunctionTemplateParamTypes={}  FunctionTemplateParamValues={}  FunctionIndex=1  FunctionTabVisible=on  FunctionTemplateParamsVisible=off  FunctionDeclTypeOptions=C[1 1]@t123@void fft_custom(adf::input_buffer< cint32, adf::extents< 256 > > && restrict sig_i, output_cascade< cacc48, void > * sig_o)  FunctionDecl=void fft_custom(adf::input_buffer< cint32, adf::extents< 256 > > && restrict sig_i, output_cascade< cacc48, void > * sig_o)  FunctionTemplateParams={}  FunctionTemplateParamsEnables={}  PortAttrs={ 'input', 'sig_i', 'adf::input_buffer< cint32, adf::extents< 256 > > & restrict', '256', '0', 'sync', ''; 'output', 'sig_o', 'output_cascade< cacc48, void > *', '', '', '', '256' }  PortAttrsEnables={'off', 'off', 'off', 'off', 'off', 'off', 'off';'off', 'off', 'off', 'off', 'off', 'off', 'on'}  SampleTime=-1  KernelHeaderFile=customFFT_casc/fft_custom.h  KernelFunction=fft_custom  KernelInitFunction=fft_custom_init  KernelSourceFile=customFFT_casc/fft_custom.cpp  KernelSearchPaths={'./customFFT_casc'}  PreProcOptions={}  blockJsonConstraints="{\"type\":\"constraint\",\"constraintType\":\"stackSize\",\"sid\":\"5811\",\"lhs\":{\"type\":\"stackSize\",\"args\":{\"type\":\"kernel\",\"name\":\"OverlapSaveFIR_11paths/custom_11copies/fft_custom7\",\"sid\":\"5811\"}},\"rhs\":{\"type\":\"value\",\"args\":{\"type\":\"evaluable\",\"expr\":\"3200\",\"value\":3200}},\"equality\":true}"
  fft_custom8 : aieBasic/AIE Kernel  KernelAllAttrs=s[12;12;9;9;19;14;21;23;21;23;24;21;15;17;12;24;26;26;26;27;28;9;21;23;23;23;24;25;14;19;19;29]@FunctionNameDeclFileNamePortNamesPortTypesPortSerializedTypesPortDirectionsPortWindowSizeEnablesPortWindowMarginEnablesPortBufferSizeEnablesPortBufferMarginEnablesPortSynchronicityEnablesPortSignalSizeEnablesPortBufferSizesPortBufferMarginsFunctionDeclFunctionTemplateSpecKindFunctionTemplateParamNamesFunctionTemplateParamKindsFunctionTemplateParamTypesFunctionTemplateParamValuesFunctionTemplateParamEnablesClassDeclClassTemplateSpecKindClassTemplateParamNamesClassTemplateParamKindsClassTemplateParamTypesClassTemplateParamValuesClassTemplateParamEnablesClassCtorDeclsClassCtorParamNamesClassCtorParamTypesClassCtorParamSerializedTypes[1 1]@C[32 1]@t10@fft_customt33@../../customFFT_casc/fft_custom.hC[2 1]@t5@sig_it5@sig_oC[2 1]@t59@adf::input_buffer< cint32, adf::extents< 256 > > & restrictt32@output_cascade< cacc48, void > *C[2 1]@t71@{Q2{R{Tadf::input_buffer{2{t{Scint32}}{t{Tadf::extents{1{t{}256}}}}}}}}t42@{P{Toutput_cascade{2{t{Scacc48}}{t{Bv}}}}}C[2 1]@t5@inputt6@outputC[2 1]@l1@l0@C[2 1]@l1@l0@C[2 1]@l1@l0@C[2 1]@l0@l0@C[2 1]@l1@l0@C[2 1]@l0@l1@C[2 1]@t3@256nC[2 1]@nnt122@void fft_custom(adf::input_buffer< cint32, adf::extents< 256 > > & restrict sig_i, output_cascade< cacc48, void > * sig_o)t4@nonee[0 1]@e[0 1]@e[0 1]@e[0 1]@e[0 1]@nne[0 1]@e[0 1]@e[0 1]@e[0 1]@e[0 1]@e[0 1]@e[0 1]@e[0 1]@e[0 1]@  PortNames={'sig_i'; 'sig_o'}  PortSerializedTypes={'{Q2{R{Tadf::input_buffer{2{t{Scint32}}{t{Tadf::extents{1{t{}256}}}}}}}}'; '{P{Toutput_cascade{2{t{Scacc48}}{t{Bv}}}}}'}  PortWindowSizes={2.560000000000000000e+02, 0.000000000000000000e+00}  PortWindowMargins={0.000000000000000000e+00, 0.000000000000000000e+00}  PortSynchronicities={'sync', 'auto'}  PortSignalSizes={0.000000000000000000e+00; 2.560000000000000000e+02}  FunctionTemplateSpecKind=none  FunctionTemplateParamNames={}  FunctionTemplateParamKinds={}  FunctionTemplateParamTypes={}  FunctionTemplateParamValues={}  FunctionIndex=1  FunctionTabVisible=on  FunctionTemplateParamsVisible=off  FunctionDeclTypeOptions=C[1 1]@t123@void fft_custom(adf::input_buffer< cint32, adf::extents< 256 > > && restrict sig_i, output_cascade< cacc48, void > * sig_o)  FunctionDecl=void fft_custom(adf::input_buffer< cint32, adf::extents< 256 > > && restrict sig_i, output_cascade< cacc48, void > * sig_o)  FunctionTemplateParams={}  FunctionTemplateParamsEnables={}  PortAttrs={ 'input', 'sig_i', 'adf::input_buffer< cint32, adf::extents< 256 > > & restrict', '256', '0', 'sync', ''; 'output', 'sig_o', 'output_cascade< cacc48, void > *', '', '', '', '256' }  PortAttrsEnables={'off', 'off', 'off', 'off', 'off', 'off', 'off';'off', 'off', 'off', 'off', 'off', 'off', 'on'}  SampleTime=-1  KernelHeaderFile=customFFT_casc/fft_custom.h  KernelFunction=fft_custom  KernelInitFunction=fft_custom_init  KernelSourceFile=customFFT_casc/fft_custom.cpp  KernelSearchPaths={'./customFFT_casc'}  PreProcOptions={}  blockJsonConstraints="{\"type\":\"constraint\",\"constraintType\":\"stackSize\",\"sid\":\"5812\",\"lhs\":{\"type\":\"stackSize\",\"args\":{\"type\":\"kernel\",\"name\":\"OverlapSaveFIR_11paths/custom_11copies/fft_custom8\",\"sid\":\"5812\"}},\"rhs\":{\"type\":\"value\",\"args\":{\"type\":\"evaluable\",\"expr\":\"3200\",\"value\":3200}},\"equality\":true}"
  fft_custom9 : aieBasic/AIE Kernel  KernelAllAttrs=s[12;12;9;9;19;14;21;23;21;23;24;21;15;17;12;24;26;26;26;27;28;9;21;23;23;23;24;25;14;19;19;29]@FunctionNameDeclFileNamePortNamesPortTypesPortSerializedTypesPortDirectionsPortWindowSizeEnablesPortWindowMarginEnablesPortBufferSizeEnablesPortBufferMarginEnablesPortSynchronicityEnablesPortSignalSizeEnablesPortBufferSizesPortBufferMarginsFunctionDeclFunctionTemplateSpecKindFunctionTemplateParamNamesFunctionTemplateParamKindsFunctionTemplateParamTypesFunctionTemplateParamValuesFunctionTemplateParamEnablesClassDeclClassTemplateSpecKindClassTemplateParamNamesClassTemplateParamKindsClassTemplateParamTypesClassTemplateParamValuesClassTemplateParamEnablesClassCtorDeclsClassCtorParamNamesClassCtorParamTypesClassCtorParamSerializedTypes[1 1]@C[32 1]@t10@fft_customt33@../../customFFT_casc/fft_custom.hC[2 1]@t5@sig_it5@sig_oC[2 1]@t59@adf::input_buffer< cint32, adf::extents< 256 > > & restrictt32@output_cascade< cacc48, void > *C[2 1]@t71@{Q2{R{Tadf::input_buffer{2{t{Scint32}}{t{Tadf::extents{1{t{}256}}}}}}}}t42@{P{Toutput_cascade{2{t{Scacc48}}{t{Bv}}}}}C[2 1]@t5@inputt6@outputC[2 1]@l1@l0@C[2 1]@l1@l0@C[2 1]@l1@l0@C[2 1]@l0@l0@C[2 1]@l1@l0@C[2 1]@l0@l1@C[2 1]@t3@256nC[2 1]@nnt122@void fft_custom(adf::input_buffer< cint32, adf::extents< 256 > > & restrict sig_i, output_cascade< cacc48, void > * sig_o)t4@nonee[0 1]@e[0 1]@e[0 1]@e[0 1]@e[0 1]@nne[0 1]@e[0 1]@e[0 1]@e[0 1]@e[0 1]@e[0 1]@e[0 1]@e[0 1]@e[0 1]@  PortNames={'sig_i'; 'sig_o'}  PortSerializedTypes={'{Q2{R{Tadf::input_buffer{2{t{Scint32}}{t{Tadf::extents{1{t{}256}}}}}}}}'; '{P{Toutput_cascade{2{t{Scacc48}}{t{Bv}}}}}'}  PortWindowSizes={2.560000000000000000e+02, 0.000000000000000000e+00}  PortWindowMargins={0.000000000000000000e+00, 0.000000000000000000e+00}  PortSynchronicities={'sync', 'auto'}  PortSignalSizes={0.000000000000000000e+00; 2.560000000000000000e+02}  FunctionTemplateSpecKind=none  FunctionTemplateParamNames={}  FunctionTemplateParamKinds={}  FunctionTemplateParamTypes={}  FunctionTemplateParamValues={}  FunctionIndex=1  FunctionTabVisible=on  FunctionTemplateParamsVisible=off  FunctionDeclTypeOptions=C[1 1]@t123@void fft_custom(adf::input_buffer< cint32, adf::extents< 256 > > && restrict sig_i, output_cascade< cacc48, void > * sig_o)  FunctionDecl=void fft_custom(adf::input_buffer< cint32, adf::extents< 256 > > && restrict sig_i, output_cascade< cacc48, void > * sig_o)  FunctionTemplateParams={}  FunctionTemplateParamsEnables={}  PortAttrs={ 'input', 'sig_i', 'adf::input_buffer< cint32, adf::extents< 256 > > & restrict', '256', '0', 'sync', ''; 'output', 'sig_o', 'output_cascade< cacc48, void > *', '', '', '', '256' }  PortAttrsEnables={'off', 'off', 'off', 'off', 'off', 'off', 'off';'off', 'off', 'off', 'off', 'off', 'off', 'on'}  SampleTime=-1  KernelHeaderFile=customFFT_casc/fft_custom.h  KernelFunction=fft_custom  KernelInitFunction=fft_custom_init  KernelSourceFile=customFFT_casc/fft_custom.cpp  KernelSearchPaths={'./customFFT_casc'}  PreProcOptions={}  blockJsonConstraints="{\"type\":\"constraint\",\"constraintType\":\"stackSize\",\"sid\":\"5847\",\"lhs\":{\"type\":\"stackSize\",\"args\":{\"type\":\"kernel\",\"name\":\"OverlapSaveFIR_11paths/custom_11copies/fft_custom9\",\"sid\":\"5847\"}},\"rhs\":{\"type\":\"value\",\"args\":{\"type\":\"evaluable\",\"expr\":\"3200\",\"value\":3200}},\"equality\":true}"
  ifft_custom : aieBasic/AIE Kernel  KernelAllAttrs=s[12;12;9;9;19;14;21;23;21;23;24;21;15;17;12;24;26;26;26;27;28;9;21;23;23;23;24;25;14;19;19;29]@FunctionNameDeclFileNamePortNamesPortTypesPortSerializedTypesPortDirectionsPortWindowSizeEnablesPortWindowMarginEnablesPortBufferSizeEnablesPortBufferMarginEnablesPortSynchronicityEnablesPortSignalSizeEnablesPortBufferSizesPortBufferMarginsFunctionDeclFunctionTemplateSpecKindFunctionTemplateParamNamesFunctionTemplateParamKindsFunctionTemplateParamTypesFunctionTemplateParamValuesFunctionTemplateParamEnablesClassDeclClassTemplateSpecKindClassTemplateParamNamesClassTemplateParamKindsClassTemplateParamTypesClassTemplateParamValuesClassTemplateParamEnablesClassCtorDeclsClassCtorParamNamesClassCtorParamTypesClassCtorParamSerializedTypes[1 1]@C[32 1]@t11@ifft_customt34@../../customFFT_casc/ifft_custom.hC[2 1]@t5@sig_it5@sig_oC[2 1]@t31@input_cascade< cacc48, void > *t60@adf::output_buffer< cint32, adf::extents< 256 > > & restrictC[2 1]@t41@{P{Tinput_cascade{2{t{Scacc48}}{t{Bv}}}}}t72@{Q2{R{Tadf::output_buffer{2{t{Scint32}}{t{Tadf::extents{1{t{}256}}}}}}}}C[2 1]@t5@inputt6@outputC[2 1]@l0@l1@C[2 1]@l0@l0@C[2 1]@l0@l1@C[2 1]@l0@l0@C[2 1]@l0@l1@C[2 1]@l0@l0@C[2 1]@nt3@256C[2 1]@nnt123@void ifft_custom(input_cascade< cacc48, void > * sig_i, adf::output_buffer< cint32, adf::extents< 256 > > & restrict sig_o)t4@nonee[0 1]@e[0 1]@e[0 1]@e[0 1]@e[0 1]@nne[0 1]@e[0 1]@e[0 1]@e[0 1]@e[0 1]@e[0 1]@e[0 1]@e[0 1]@e[0 1]@  PortNames={'sig_i'; 'sig_o'}  PortSerializedTypes={'{P{Tinput_cascade{2{t{Scacc48}}{t{Bv}}}}}'; '{Q2{R{Tadf::output_buffer{2{t{Scint32}}{t{Tadf::extents{1{t{}256}}}}}}}}'}  PortWindowSizes={0.000000000000000000e+00, 2.560000000000000000e+02}  PortWindowMargins={0.000000000000000000e+00, 0.000000000000000000e+00}  PortSynchronicities={'auto', 'sync'}  PortSignalSizes={0.000000000000000000e+00; 0.000000000000000000e+00}  FunctionTemplateSpecKind=none  FunctionTemplateParamNames={}  FunctionTemplateParamKinds={}  FunctionTemplateParamTypes={}  FunctionTemplateParamValues={}  FunctionIndex=1  FunctionTabVisible=on  FunctionTemplateParamsVisible=off  FunctionDeclTypeOptions=C[1 1]@t124@void ifft_custom(input_cascade< cacc48, void > * sig_i, adf::output_buffer< cint32, adf::extents< 256 > > && restrict sig_o)  FunctionDecl=void ifft_custom(input_cascade< cacc48, void > * sig_i, adf::output_buffer< cint32, adf::extents< 256 > > && restrict sig_o)  FunctionTemplateParams={}  FunctionTemplateParamsEnables={}  PortAttrs={ 'input', 'sig_i', 'input_cascade< cacc48, void > *', '', '', '', ''; 'output', 'sig_o', 'adf::output_buffer< cint32, adf::extents< 256 > > & restrict', '256', '', 'sync', '' }  PortAttrsEnables={'off', 'off', 'off', 'off', 'off', 'off', 'off';'off', 'off', 'off', 'off', 'off', 'off', 'off'}  SampleTime=-1  KernelHeaderFile=customFFT_casc/ifft_custom.h  KernelFunction=ifft_custom  KernelInitFunction=ifft_custom_init  KernelSourceFile=customFFT_casc/ifft_custom.cpp  KernelSearchPaths={'./customFFT_casc'}  PreProcOptions={}  blockJsonConstraints="{\"type\":\"constraint\",\"constraintType\":\"stackSize\",\"sid\":\"5824\",\"lhs\":{\"type\":\"stackSize\",\"args\":{\"type\":\"kernel\",\"name\":\"OverlapSaveFIR_11paths/custom_11copies/ifft_custom\",\"sid\":\"5824\"}},\"rhs\":{\"type\":\"value\",\"args\":{\"type\":\"evaluable\",\"expr\":\"4200\",\"value\":4200}},\"equality\":true}"
  ifft_custom1 : aieBasic/AIE Kernel  KernelAllAttrs=s[12;12;9;9;19;14;21;23;21;23;24;21;15;17;12;24;26;26;26;27;28;9;21;23;23;23;24;25;14;19;19;29]@FunctionNameDeclFileNamePortNamesPortTypesPortSerializedTypesPortDirectionsPortWindowSizeEnablesPortWindowMarginEnablesPortBufferSizeEnablesPortBufferMarginEnablesPortSynchronicityEnablesPortSignalSizeEnablesPortBufferSizesPortBufferMarginsFunctionDeclFunctionTemplateSpecKindFunctionTemplateParamNamesFunctionTemplateParamKindsFunctionTemplateParamTypesFunctionTemplateParamValuesFunctionTemplateParamEnablesClassDeclClassTemplateSpecKindClassTemplateParamNamesClassTemplateParamKindsClassTemplateParamTypesClassTemplateParamValuesClassTemplateParamEnablesClassCtorDeclsClassCtorParamNamesClassCtorParamTypesClassCtorParamSerializedTypes[1 1]@C[32 1]@t11@ifft_customt34@../../customFFT_casc/ifft_custom.hC[2 1]@t5@sig_it5@sig_oC[2 1]@t31@input_cascade< cacc48, void > *t60@adf::output_buffer< cint32, adf::extents< 256 > > & restrictC[2 1]@t41@{P{Tinput_cascade{2{t{Scacc48}}{t{Bv}}}}}t72@{Q2{R{Tadf::output_buffer{2{t{Scint32}}{t{Tadf::extents{1{t{}256}}}}}}}}C[2 1]@t5@inputt6@outputC[2 1]@l0@l1@C[2 1]@l0@l0@C[2 1]@l0@l1@C[2 1]@l0@l0@C[2 1]@l0@l1@C[2 1]@l0@l0@C[2 1]@nt3@256C[2 1]@nnt123@void ifft_custom(input_cascade< cacc48, void > * sig_i, adf::output_buffer< cint32, adf::extents< 256 > > & restrict sig_o)t4@nonee[0 1]@e[0 1]@e[0 1]@e[0 1]@e[0 1]@nne[0 1]@e[0 1]@e[0 1]@e[0 1]@e[0 1]@e[0 1]@e[0 1]@e[0 1]@e[0 1]@  PortNames={'sig_i'; 'sig_o'}  PortSerializedTypes={'{P{Tinput_cascade{2{t{Scacc48}}{t{Bv}}}}}'; '{Q2{R{Tadf::output_buffer{2{t{Scint32}}{t{Tadf::extents{1{t{}256}}}}}}}}'}  PortWindowSizes={0.000000000000000000e+00, 2.560000000000000000e+02}  PortWindowMargins={0.000000000000000000e+00, 0.000000000000000000e+00}  PortSynchronicities={'auto', 'sync'}  PortSignalSizes={0.000000000000000000e+00; 0.000000000000000000e+00}  FunctionTemplateSpecKind=none  FunctionTemplateParamNames={}  FunctionTemplateParamKinds={}  FunctionTemplateParamTypes={}  FunctionTemplateParamValues={}  FunctionIndex=1  FunctionTabVisible=on  FunctionTemplateParamsVisible=off  FunctionDeclTypeOptions=C[1 1]@t124@void ifft_custom(input_cascade< cacc48, void > * sig_i, adf::output_buffer< cint32, adf::extents< 256 > > && restrict sig_o)  FunctionDecl=void ifft_custom(input_cascade< cacc48, void > * sig_i, adf::output_buffer< cint32, adf::extents< 256 > > && restrict sig_o)  FunctionTemplateParams={}  FunctionTemplateParamsEnables={}  PortAttrs={ 'input', 'sig_i', 'input_cascade< cacc48, void > *', '', '', '', ''; 'output', 'sig_o', 'adf::output_buffer< cint32, adf::extents< 256 > > & restrict', '256', '', 'sync', '' }  PortAttrsEnables={'off', 'off', 'off', 'off', 'off', 'off', 'off';'off', 'off', 'off', 'off', 'off', 'off', 'off'}  SampleTime=-1  KernelHeaderFile=customFFT_casc/ifft_custom.h  KernelFunction=ifft_custom  KernelInitFunction=ifft_custom_init  KernelSourceFile=customFFT_casc/ifft_custom.cpp  KernelSearchPaths={'./customFFT_casc'}  PreProcOptions={}  blockJsonConstraints="{\"type\":\"constraint\",\"constraintType\":\"stackSize\",\"sid\":\"5825\",\"lhs\":{\"type\":\"stackSize\",\"args\":{\"type\":\"kernel\",\"name\":\"OverlapSaveFIR_11paths/custom_11copies/ifft_custom1\",\"sid\":\"5825\"}},\"rhs\":{\"type\":\"value\",\"args\":{\"type\":\"evaluable\",\"expr\":\"4200\",\"value\":4200}},\"equality\":true}"
  ifft_custom10 : aieBasic/AIE Kernel  KernelAllAttrs=s[12;12;9;9;19;14;21;23;21;23;24;21;15;17;12;24;26;26;26;27;28;9;21;23;23;23;24;25;14;19;19;29]@FunctionNameDeclFileNamePortNamesPortTypesPortSerializedTypesPortDirectionsPortWindowSizeEnablesPortWindowMarginEnablesPortBufferSizeEnablesPortBufferMarginEnablesPortSynchronicityEnablesPortSignalSizeEnablesPortBufferSizesPortBufferMarginsFunctionDeclFunctionTemplateSpecKindFunctionTemplateParamNamesFunctionTemplateParamKindsFunctionTemplateParamTypesFunctionTemplateParamValuesFunctionTemplateParamEnablesClassDeclClassTemplateSpecKindClassTemplateParamNamesClassTemplateParamKindsClassTemplateParamTypesClassTemplateParamValuesClassTemplateParamEnablesClassCtorDeclsClassCtorParamNamesClassCtorParamTypesClassCtorParamSerializedTypes[1 1]@C[32 1]@t11@ifft_customt34@../../customFFT_casc/ifft_custom.hC[2 1]@t5@sig_it5@sig_oC[2 1]@t31@input_cascade< cacc48, void > *t60@adf::output_buffer< cint32, adf::extents< 256 > > & restrictC[2 1]@t41@{P{Tinput_cascade{2{t{Scacc48}}{t{Bv}}}}}t72@{Q2{R{Tadf::output_buffer{2{t{Scint32}}{t{Tadf::extents{1{t{}256}}}}}}}}C[2 1]@t5@inputt6@outputC[2 1]@l0@l1@C[2 1]@l0@l0@C[2 1]@l0@l1@C[2 1]@l0@l0@C[2 1]@l0@l1@C[2 1]@l0@l0@C[2 1]@nt3@256C[2 1]@nnt123@void ifft_custom(input_cascade< cacc48, void > * sig_i, adf::output_buffer< cint32, adf::extents< 256 > > & restrict sig_o)t4@nonee[0 1]@e[0 1]@e[0 1]@e[0 1]@e[0 1]@nne[0 1]@e[0 1]@e[0 1]@e[0 1]@e[0 1]@e[0 1]@e[0 1]@e[0 1]@e[0 1]@  PortNames={'sig_i'; 'sig_o'}  PortSerializedTypes={'{P{Tinput_cascade{2{t{Scacc48}}{t{Bv}}}}}'; '{Q2{R{Tadf::output_buffer{2{t{Scint32}}{t{Tadf::extents{1{t{}256}}}}}}}}'}  PortWindowSizes={0.000000000000000000e+00, 2.560000000000000000e+02}  PortWindowMargins={0.000000000000000000e+00, 0.000000000000000000e+00}  PortSynchronicities={'auto', 'sync'}  PortSignalSizes={0.000000000000000000e+00; 0.000000000000000000e+00}  FunctionTemplateSpecKind=none  FunctionTemplateParamNames={}  FunctionTemplateParamKinds={}  FunctionTemplateParamTypes={}  FunctionTemplateParamValues={}  FunctionIndex=1  FunctionTabVisible=on  FunctionTemplateParamsVisible=off  FunctionDeclTypeOptions=C[1 1]@t124@void ifft_custom(input_cascade< cacc48, void > * sig_i, adf::output_buffer< cint32, adf::extents< 256 > > && restrict sig_o)  FunctionDecl=void ifft_custom(input_cascade< cacc48, void > * sig_i, adf::output_buffer< cint32, adf::extents< 256 > > && restrict sig_o)  FunctionTemplateParams={}  FunctionTemplateParamsEnables={}  PortAttrs={ 'input', 'sig_i', 'input_cascade< cacc48, void > *', '', '', '', ''; 'output', 'sig_o', 'adf::output_buffer< cint32, adf::extents< 256 > > & restrict', '256', '', 'sync', '' }  PortAttrsEnables={'off', 'off', 'off', 'off', 'off', 'off', 'off';'off', 'off', 'off', 'off', 'off', 'off', 'off'}  SampleTime=-1  KernelHeaderFile=customFFT_casc/ifft_custom.h  KernelFunction=ifft_custom  KernelInitFunction=ifft_custom_init  KernelSourceFile=customFFT_casc/ifft_custom.cpp  KernelSearchPaths={'./customFFT_casc'}  PreProcOptions={}  blockJsonConstraints="{\"type\":\"constraint\",\"constraintType\":\"stackSize\",\"sid\":\"5873\",\"lhs\":{\"type\":\"stackSize\",\"args\":{\"type\":\"kernel\",\"name\":\"OverlapSaveFIR_11paths/custom_11copies/ifft_custom10\",\"sid\":\"5873\"}},\"rhs\":{\"type\":\"value\",\"args\":{\"type\":\"evaluable\",\"expr\":\"4200\",\"value\":4200}},\"equality\":true}"
  ifft_custom2 : aieBasic/AIE Kernel  KernelAllAttrs=s[12;12;9;9;19;14;21;23;21;23;24;21;15;17;12;24;26;26;26;27;28;9;21;23;23;23;24;25;14;19;19;29]@FunctionNameDeclFileNamePortNamesPortTypesPortSerializedTypesPortDirectionsPortWindowSizeEnablesPortWindowMarginEnablesPortBufferSizeEnablesPortBufferMarginEnablesPortSynchronicityEnablesPortSignalSizeEnablesPortBufferSizesPortBufferMarginsFunctionDeclFunctionTemplateSpecKindFunctionTemplateParamNamesFunctionTemplateParamKindsFunctionTemplateParamTypesFunctionTemplateParamValuesFunctionTemplateParamEnablesClassDeclClassTemplateSpecKindClassTemplateParamNamesClassTemplateParamKindsClassTemplateParamTypesClassTemplateParamValuesClassTemplateParamEnablesClassCtorDeclsClassCtorParamNamesClassCtorParamTypesClassCtorParamSerializedTypes[1 1]@C[32 1]@t11@ifft_customt34@../../customFFT_casc/ifft_custom.hC[2 1]@t5@sig_it5@sig_oC[2 1]@t31@input_cascade< cacc48, void > *t60@adf::output_buffer< cint32, adf::extents< 256 > > & restrictC[2 1]@t41@{P{Tinput_cascade{2{t{Scacc48}}{t{Bv}}}}}t72@{Q2{R{Tadf::output_buffer{2{t{Scint32}}{t{Tadf::extents{1{t{}256}}}}}}}}C[2 1]@t5@inputt6@outputC[2 1]@l0@l1@C[2 1]@l0@l0@C[2 1]@l0@l1@C[2 1]@l0@l0@C[2 1]@l0@l1@C[2 1]@l0@l0@C[2 1]@nt3@256C[2 1]@nnt123@void ifft_custom(input_cascade< cacc48, void > * sig_i, adf::output_buffer< cint32, adf::extents< 256 > > & restrict sig_o)t4@nonee[0 1]@e[0 1]@e[0 1]@e[0 1]@e[0 1]@nne[0 1]@e[0 1]@e[0 1]@e[0 1]@e[0 1]@e[0 1]@e[0 1]@e[0 1]@e[0 1]@  PortNames={'sig_i'; 'sig_o'}  PortSerializedTypes={'{P{Tinput_cascade{2{t{Scacc48}}{t{Bv}}}}}'; '{Q2{R{Tadf::output_buffer{2{t{Scint32}}{t{Tadf::extents{1{t{}256}}}}}}}}'}  PortWindowSizes={0.000000000000000000e+00, 2.560000000000000000e+02}  PortWindowMargins={0.000000000000000000e+00, 0.000000000000000000e+00}  PortSynchronicities={'auto', 'sync'}  PortSignalSizes={0.000000000000000000e+00; 0.000000000000000000e+00}  FunctionTemplateSpecKind=none  FunctionTemplateParamNames={}  FunctionTemplateParamKinds={}  FunctionTemplateParamTypes={}  FunctionTemplateParamValues={}  FunctionIndex=1  FunctionTabVisible=on  FunctionTemplateParamsVisible=off  FunctionDeclTypeOptions=C[1 1]@t124@void ifft_custom(input_cascade< cacc48, void > * sig_i, adf::output_buffer< cint32, adf::extents< 256 > > && restrict sig_o)  FunctionDecl=void ifft_custom(input_cascade< cacc48, void > * sig_i, adf::output_buffer< cint32, adf::extents< 256 > > && restrict sig_o)  FunctionTemplateParams={}  FunctionTemplateParamsEnables={}  PortAttrs={ 'input', 'sig_i', 'input_cascade< cacc48, void > *', '', '', '', ''; 'output', 'sig_o', 'adf::output_buffer< cint32, adf::extents< 256 > > & restrict', '256', '', 'sync', '' }  PortAttrsEnables={'off', 'off', 'off', 'off', 'off', 'off', 'off';'off', 'off', 'off', 'off', 'off', 'off', 'off'}  SampleTime=-1  KernelHeaderFile=customFFT_casc/ifft_custom.h  KernelFunction=ifft_custom  KernelInitFunction=ifft_custom_init  KernelSourceFile=customFFT_casc/ifft_custom.cpp  KernelSearchPaths={'./customFFT_casc'}  PreProcOptions={}  blockJsonConstraints="{\"type\":\"constraint\",\"constraintType\":\"stackSize\",\"sid\":\"5826\",\"lhs\":{\"type\":\"stackSize\",\"args\":{\"type\":\"kernel\",\"name\":\"OverlapSaveFIR_11paths/custom_11copies/ifft_custom2\",\"sid\":\"5826\"}},\"rhs\":{\"type\":\"value\",\"args\":{\"type\":\"evaluable\",\"expr\":\"4200\",\"value\":4200}},\"equality\":true}"
  ifft_custom3 : aieBasic/AIE Kernel  KernelAllAttrs=s[12;12;9;9;19;14;21;23;21;23;24;21;15;17;12;24;26;26;26;27;28;9;21;23;23;23;24;25;14;19;19;29]@FunctionNameDeclFileNamePortNamesPortTypesPortSerializedTypesPortDirectionsPortWindowSizeEnablesPortWindowMarginEnablesPortBufferSizeEnablesPortBufferMarginEnablesPortSynchronicityEnablesPortSignalSizeEnablesPortBufferSizesPortBufferMarginsFunctionDeclFunctionTemplateSpecKindFunctionTemplateParamNamesFunctionTemplateParamKindsFunctionTemplateParamTypesFunctionTemplateParamValuesFunctionTemplateParamEnablesClassDeclClassTemplateSpecKindClassTemplateParamNamesClassTemplateParamKindsClassTemplateParamTypesClassTemplateParamValuesClassTemplateParamEnablesClassCtorDeclsClassCtorParamNamesClassCtorParamTypesClassCtorParamSerializedTypes[1 1]@C[32 1]@t11@ifft_customt34@../../customFFT_casc/ifft_custom.hC[2 1]@t5@sig_it5@sig_oC[2 1]@t31@input_cascade< cacc48, void > *t60@adf::output_buffer< cint32, adf::extents< 256 > > & restrictC[2 1]@t41@{P{Tinput_cascade{2{t{Scacc48}}{t{Bv}}}}}t72@{Q2{R{Tadf::output_buffer{2{t{Scint32}}{t{Tadf::extents{1{t{}256}}}}}}}}C[2 1]@t5@inputt6@outputC[2 1]@l0@l1@C[2 1]@l0@l0@C[2 1]@l0@l1@C[2 1]@l0@l0@C[2 1]@l0@l1@C[2 1]@l0@l0@C[2 1]@nt3@256C[2 1]@nnt123@void ifft_custom(input_cascade< cacc48, void > * sig_i, adf::output_buffer< cint32, adf::extents< 256 > > & restrict sig_o)t4@nonee[0 1]@e[0 1]@e[0 1]@e[0 1]@e[0 1]@nne[0 1]@e[0 1]@e[0 1]@e[0 1]@e[0 1]@e[0 1]@e[0 1]@e[0 1]@e[0 1]@  PortNames={'sig_i'; 'sig_o'}  PortSerializedTypes={'{P{Tinput_cascade{2{t{Scacc48}}{t{Bv}}}}}'; '{Q2{R{Tadf::output_buffer{2{t{Scint32}}{t{Tadf::extents{1{t{}256}}}}}}}}'}  PortWindowSizes={0.000000000000000000e+00, 2.560000000000000000e+02}  PortWindowMargins={0.000000000000000000e+00, 0.000000000000000000e+00}  PortSynchronicities={'auto', 'sync'}  PortSignalSizes={0.000000000000000000e+00; 0.000000000000000000e+00}  FunctionTemplateSpecKind=none  FunctionTemplateParamNames={}  FunctionTemplateParamKinds={}  FunctionTemplateParamTypes={}  FunctionTemplateParamValues={}  FunctionIndex=1  FunctionTabVisible=on  FunctionTemplateParamsVisible=off  FunctionDeclTypeOptions=C[1 1]@t124@void ifft_custom(input_cascade< cacc48, void > * sig_i, adf::output_buffer< cint32, adf::extents< 256 > > && restrict sig_o)  FunctionDecl=void ifft_custom(input_cascade< cacc48, void > * sig_i, adf::output_buffer< cint32, adf::extents< 256 > > && restrict sig_o)  FunctionTemplateParams={}  FunctionTemplateParamsEnables={}  PortAttrs={ 'input', 'sig_i', 'input_cascade< cacc48, void > *', '', '', '', ''; 'output', 'sig_o', 'adf::output_buffer< cint32, adf::extents< 256 > > & restrict', '256', '', 'sync', '' }  PortAttrsEnables={'off', 'off', 'off', 'off', 'off', 'off', 'off';'off', 'off', 'off', 'off', 'off', 'off', 'off'}  SampleTime=-1  KernelHeaderFile=customFFT_casc/ifft_custom.h  KernelFunction=ifft_custom  KernelInitFunction=ifft_custom_init  KernelSourceFile=customFFT_casc/ifft_custom.cpp  KernelSearchPaths={'./customFFT_casc'}  PreProcOptions={}  blockJsonConstraints="{\"type\":\"constraint\",\"constraintType\":\"stackSize\",\"sid\":\"5827\",\"lhs\":{\"type\":\"stackSize\",\"args\":{\"type\":\"kernel\",\"name\":\"OverlapSaveFIR_11paths/custom_11copies/ifft_custom3\",\"sid\":\"5827\"}},\"rhs\":{\"type\":\"value\",\"args\":{\"type\":\"evaluable\",\"expr\":\"4200\",\"value\":4200}},\"equality\":true}"
  ifft_custom4 : aieBasic/AIE Kernel  KernelAllAttrs=s[12;12;9;9;19;14;21;23;21;23;24;21;15;17;12;24;26;26;26;27;28;9;21;23;23;23;24;25;14;19;19;29]@FunctionNameDeclFileNamePortNamesPortTypesPortSerializedTypesPortDirectionsPortWindowSizeEnablesPortWindowMarginEnablesPortBufferSizeEnablesPortBufferMarginEnablesPortSynchronicityEnablesPortSignalSizeEnablesPortBufferSizesPortBufferMarginsFunctionDeclFunctionTemplateSpecKindFunctionTemplateParamNamesFunctionTemplateParamKindsFunctionTemplateParamTypesFunctionTemplateParamValuesFunctionTemplateParamEnablesClassDeclClassTemplateSpecKindClassTemplateParamNamesClassTemplateParamKindsClassTemplateParamTypesClassTemplateParamValuesClassTemplateParamEnablesClassCtorDeclsClassCtorParamNamesClassCtorParamTypesClassCtorParamSerializedTypes[1 1]@C[32 1]@t11@ifft_customt34@../../customFFT_casc/ifft_custom.hC[2 1]@t5@sig_it5@sig_oC[2 1]@t31@input_cascade< cacc48, void > *t60@adf::output_buffer< cint32, adf::extents< 256 > > & restrictC[2 1]@t41@{P{Tinput_cascade{2{t{Scacc48}}{t{Bv}}}}}t72@{Q2{R{Tadf::output_buffer{2{t{Scint32}}{t{Tadf::extents{1{t{}256}}}}}}}}C[2 1]@t5@inputt6@outputC[2 1]@l0@l1@C[2 1]@l0@l0@C[2 1]@l0@l1@C[2 1]@l0@l0@C[2 1]@l0@l1@C[2 1]@l0@l0@C[2 1]@nt3@256C[2 1]@nnt123@void ifft_custom(input_cascade< cacc48, void > * sig_i, adf::output_buffer< cint32, adf::extents< 256 > > & restrict sig_o)t4@nonee[0 1]@e[0 1]@e[0 1]@e[0 1]@e[0 1]@nne[0 1]@e[0 1]@e[0 1]@e[0 1]@e[0 1]@e[0 1]@e[0 1]@e[0 1]@e[0 1]@  PortNames={'sig_i'; 'sig_o'}  PortSerializedTypes={'{P{Tinput_cascade{2{t{Scacc48}}{t{Bv}}}}}'; '{Q2{R{Tadf::output_buffer{2{t{Scint32}}{t{Tadf::extents{1{t{}256}}}}}}}}'}  PortWindowSizes={0.000000000000000000e+00, 2.560000000000000000e+02}  PortWindowMargins={0.000000000000000000e+00, 0.000000000000000000e+00}  PortSynchronicities={'auto', 'sync'}  PortSignalSizes={0.000000000000000000e+00; 0.000000000000000000e+00}  FunctionTemplateSpecKind=none  FunctionTemplateParamNames={}  FunctionTemplateParamKinds={}  FunctionTemplateParamTypes={}  FunctionTemplateParamValues={}  FunctionIndex=1  FunctionTabVisible=on  FunctionTemplateParamsVisible=off  FunctionDeclTypeOptions=C[1 1]@t124@void ifft_custom(input_cascade< cacc48, void > * sig_i, adf::output_buffer< cint32, adf::extents< 256 > > && restrict sig_o)  FunctionDecl=void ifft_custom(input_cascade< cacc48, void > * sig_i, adf::output_buffer< cint32, adf::extents< 256 > > && restrict sig_o)  FunctionTemplateParams={}  FunctionTemplateParamsEnables={}  PortAttrs={ 'input', 'sig_i', 'input_cascade< cacc48, void > *', '', '', '', ''; 'output', 'sig_o', 'adf::output_buffer< cint32, adf::extents< 256 > > & restrict', '256', '', 'sync', '' }  PortAttrsEnables={'off', 'off', 'off', 'off', 'off', 'off', 'off';'off', 'off', 'off', 'off', 'off', 'off', 'off'}  SampleTime=-1  KernelHeaderFile=customFFT_casc/ifft_custom.h  KernelFunction=ifft_custom  KernelInitFunction=ifft_custom_init  KernelSourceFile=customFFT_casc/ifft_custom.cpp  KernelSearchPaths={'./customFFT_casc'}  PreProcOptions={}  blockJsonConstraints="{\"type\":\"constraint\",\"constraintType\":\"stackSize\",\"sid\":\"5828\",\"lhs\":{\"type\":\"stackSize\",\"args\":{\"type\":\"kernel\",\"name\":\"OverlapSaveFIR_11paths/custom_11copies/ifft_custom4\",\"sid\":\"5828\"}},\"rhs\":{\"type\":\"value\",\"args\":{\"type\":\"evaluable\",\"expr\":\"4200\",\"value\":4200}},\"equality\":true}"
  ifft_custom5 : aieBasic/AIE Kernel  KernelAllAttrs=s[12;12;9;9;19;14;21;23;21;23;24;21;15;17;12;24;26;26;26;27;28;9;21;23;23;23;24;25;14;19;19;29]@FunctionNameDeclFileNamePortNamesPortTypesPortSerializedTypesPortDirectionsPortWindowSizeEnablesPortWindowMarginEnablesPortBufferSizeEnablesPortBufferMarginEnablesPortSynchronicityEnablesPortSignalSizeEnablesPortBufferSizesPortBufferMarginsFunctionDeclFunctionTemplateSpecKindFunctionTemplateParamNamesFunctionTemplateParamKindsFunctionTemplateParamTypesFunctionTemplateParamValuesFunctionTemplateParamEnablesClassDeclClassTemplateSpecKindClassTemplateParamNamesClassTemplateParamKindsClassTemplateParamTypesClassTemplateParamValuesClassTemplateParamEnablesClassCtorDeclsClassCtorParamNamesClassCtorParamTypesClassCtorParamSerializedTypes[1 1]@C[32 1]@t11@ifft_customt34@../../customFFT_casc/ifft_custom.hC[2 1]@t5@sig_it5@sig_oC[2 1]@t31@input_cascade< cacc48, void > *t60@adf::output_buffer< cint32, adf::extents< 256 > > & restrictC[2 1]@t41@{P{Tinput_cascade{2{t{Scacc48}}{t{Bv}}}}}t72@{Q2{R{Tadf::output_buffer{2{t{Scint32}}{t{Tadf::extents{1{t{}256}}}}}}}}C[2 1]@t5@inputt6@outputC[2 1]@l0@l1@C[2 1]@l0@l0@C[2 1]@l0@l1@C[2 1]@l0@l0@C[2 1]@l0@l1@C[2 1]@l0@l0@C[2 1]@nt3@256C[2 1]@nnt123@void ifft_custom(input_cascade< cacc48, void > * sig_i, adf::output_buffer< cint32, adf::extents< 256 > > & restrict sig_o)t4@nonee[0 1]@e[0 1]@e[0 1]@e[0 1]@e[0 1]@nne[0 1]@e[0 1]@e[0 1]@e[0 1]@e[0 1]@e[0 1]@e[0 1]@e[0 1]@e[0 1]@  PortNames={'sig_i'; 'sig_o'}  PortSerializedTypes={'{P{Tinput_cascade{2{t{Scacc48}}{t{Bv}}}}}'; '{Q2{R{Tadf::output_buffer{2{t{Scint32}}{t{Tadf::extents{1{t{}256}}}}}}}}'}  PortWindowSizes={0.000000000000000000e+00, 2.560000000000000000e+02}  PortWindowMargins={0.000000000000000000e+00, 0.000000000000000000e+00}  PortSynchronicities={'auto', 'sync'}  PortSignalSizes={0.000000000000000000e+00; 0.000000000000000000e+00}  FunctionTemplateSpecKind=none  FunctionTemplateParamNames={}  FunctionTemplateParamKinds={}  FunctionTemplateParamTypes={}  FunctionTemplateParamValues={}  FunctionIndex=1  FunctionTabVisible=on  FunctionTemplateParamsVisible=off  FunctionDeclTypeOptions=C[1 1]@t124@void ifft_custom(input_cascade< cacc48, void > * sig_i, adf::output_buffer< cint32, adf::extents< 256 > > && restrict sig_o)  FunctionDecl=void ifft_custom(input_cascade< cacc48, void > * sig_i, adf::output_buffer< cint32, adf::extents< 256 > > && restrict sig_o)  FunctionTemplateParams={}  FunctionTemplateParamsEnables={}  PortAttrs={ 'input', 'sig_i', 'input_cascade< cacc48, void > *', '', '', '', ''; 'output', 'sig_o', 'adf::output_buffer< cint32, adf::extents< 256 > > & restrict', '256', '', 'sync', '' }  PortAttrsEnables={'off', 'off', 'off', 'off', 'off', 'off', 'off';'off', 'off', 'off', 'off', 'off', 'off', 'off'}  SampleTime=-1  KernelHeaderFile=customFFT_casc/ifft_custom.h  KernelFunction=ifft_custom  KernelInitFunction=ifft_custom_init  KernelSourceFile=customFFT_casc/ifft_custom.cpp  KernelSearchPaths={'./customFFT_casc'}  PreProcOptions={}  blockJsonConstraints="{\"type\":\"constraint\",\"constraintType\":\"stackSize\",\"sid\":\"5829\",\"lhs\":{\"type\":\"stackSize\",\"args\":{\"type\":\"kernel\",\"name\":\"OverlapSaveFIR_11paths/custom_11copies/ifft_custom5\",\"sid\":\"5829\"}},\"rhs\":{\"type\":\"value\",\"args\":{\"type\":\"evaluable\",\"expr\":\"4200\",\"value\":4200}},\"equality\":true}"
  ifft_custom6 : aieBasic/AIE Kernel  KernelAllAttrs=s[12;12;9;9;19;14;21;23;21;23;24;21;15;17;12;24;26;26;26;27;28;9;21;23;23;23;24;25;14;19;19;29]@FunctionNameDeclFileNamePortNamesPortTypesPortSerializedTypesPortDirectionsPortWindowSizeEnablesPortWindowMarginEnablesPortBufferSizeEnablesPortBufferMarginEnablesPortSynchronicityEnablesPortSignalSizeEnablesPortBufferSizesPortBufferMarginsFunctionDeclFunctionTemplateSpecKindFunctionTemplateParamNamesFunctionTemplateParamKindsFunctionTemplateParamTypesFunctionTemplateParamValuesFunctionTemplateParamEnablesClassDeclClassTemplateSpecKindClassTemplateParamNamesClassTemplateParamKindsClassTemplateParamTypesClassTemplateParamValuesClassTemplateParamEnablesClassCtorDeclsClassCtorParamNamesClassCtorParamTypesClassCtorParamSerializedTypes[1 1]@C[32 1]@t11@ifft_customt34@../../customFFT_casc/ifft_custom.hC[2 1]@t5@sig_it5@sig_oC[2 1]@t31@input_cascade< cacc48, void > *t60@adf::output_buffer< cint32, adf::extents< 256 > > & restrictC[2 1]@t41@{P{Tinput_cascade{2{t{Scacc48}}{t{Bv}}}}}t72@{Q2{R{Tadf::output_buffer{2{t{Scint32}}{t{Tadf::extents{1{t{}256}}}}}}}}C[2 1]@t5@inputt6@outputC[2 1]@l0@l1@C[2 1]@l0@l0@C[2 1]@l0@l1@C[2 1]@l0@l0@C[2 1]@l0@l1@C[2 1]@l0@l0@C[2 1]@nt3@256C[2 1]@nnt123@void ifft_custom(input_cascade< cacc48, void > * sig_i, adf::output_buffer< cint32, adf::extents< 256 > > & restrict sig_o)t4@nonee[0 1]@e[0 1]@e[0 1]@e[0 1]@e[0 1]@nne[0 1]@e[0 1]@e[0 1]@e[0 1]@e[0 1]@e[0 1]@e[0 1]@e[0 1]@e[0 1]@  PortNames={'sig_i'; 'sig_o'}  PortSerializedTypes={'{P{Tinput_cascade{2{t{Scacc48}}{t{Bv}}}}}'; '{Q2{R{Tadf::output_buffer{2{t{Scint32}}{t{Tadf::extents{1{t{}256}}}}}}}}'}  PortWindowSizes={0.000000000000000000e+00, 2.560000000000000000e+02}  PortWindowMargins={0.000000000000000000e+00, 0.000000000000000000e+00}  PortSynchronicities={'auto', 'sync'}  PortSignalSizes={0.000000000000000000e+00; 0.000000000000000000e+00}  FunctionTemplateSpecKind=none  FunctionTemplateParamNames={}  FunctionTemplateParamKinds={}  FunctionTemplateParamTypes={}  FunctionTemplateParamValues={}  FunctionIndex=1  FunctionTabVisible=on  FunctionTemplateParamsVisible=off  FunctionDeclTypeOptions=C[1 1]@t124@void ifft_custom(input_cascade< cacc48, void > * sig_i, adf::output_buffer< cint32, adf::extents< 256 > > && restrict sig_o)  FunctionDecl=void ifft_custom(input_cascade< cacc48, void > * sig_i, adf::output_buffer< cint32, adf::extents< 256 > > && restrict sig_o)  FunctionTemplateParams={}  FunctionTemplateParamsEnables={}  PortAttrs={ 'input', 'sig_i', 'input_cascade< cacc48, void > *', '', '', '', ''; 'output', 'sig_o', 'adf::output_buffer< cint32, adf::extents< 256 > > & restrict', '256', '', 'sync', '' }  PortAttrsEnables={'off', 'off', 'off', 'off', 'off', 'off', 'off';'off', 'off', 'off', 'off', 'off', 'off', 'off'}  SampleTime=-1  KernelHeaderFile=customFFT_casc/ifft_custom.h  KernelFunction=ifft_custom  KernelInitFunction=ifft_custom_init  KernelSourceFile=customFFT_casc/ifft_custom.cpp  KernelSearchPaths={'./customFFT_casc'}  PreProcOptions={}  blockJsonConstraints="{\"type\":\"constraint\",\"constraintType\":\"stackSize\",\"sid\":\"5830\",\"lhs\":{\"type\":\"stackSize\",\"args\":{\"type\":\"kernel\",\"name\":\"OverlapSaveFIR_11paths/custom_11copies/ifft_custom6\",\"sid\":\"5830\"}},\"rhs\":{\"type\":\"value\",\"args\":{\"type\":\"evaluable\",\"expr\":\"4200\",\"value\":4200}},\"equality\":true}"
  ifft_custom7 : aieBasic/AIE Kernel  KernelAllAttrs=s[12;12;9;9;19;14;21;23;21;23;24;21;15;17;12;24;26;26;26;27;28;9;21;23;23;23;24;25;14;19;19;29]@FunctionNameDeclFileNamePortNamesPortTypesPortSerializedTypesPortDirectionsPortWindowSizeEnablesPortWindowMarginEnablesPortBufferSizeEnablesPortBufferMarginEnablesPortSynchronicityEnablesPortSignalSizeEnablesPortBufferSizesPortBufferMarginsFunctionDeclFunctionTemplateSpecKindFunctionTemplateParamNamesFunctionTemplateParamKindsFunctionTemplateParamTypesFunctionTemplateParamValuesFunctionTemplateParamEnablesClassDeclClassTemplateSpecKindClassTemplateParamNamesClassTemplateParamKindsClassTemplateParamTypesClassTemplateParamValuesClassTemplateParamEnablesClassCtorDeclsClassCtorParamNamesClassCtorParamTypesClassCtorParamSerializedTypes[1 1]@C[32 1]@t11@ifft_customt34@../../customFFT_casc/ifft_custom.hC[2 1]@t5@sig_it5@sig_oC[2 1]@t31@input_cascade< cacc48, void > *t60@adf::output_buffer< cint32, adf::extents< 256 > > & restrictC[2 1]@t41@{P{Tinput_cascade{2{t{Scacc48}}{t{Bv}}}}}t72@{Q2{R{Tadf::output_buffer{2{t{Scint32}}{t{Tadf::extents{1{t{}256}}}}}}}}C[2 1]@t5@inputt6@outputC[2 1]@l0@l1@C[2 1]@l0@l0@C[2 1]@l0@l1@C[2 1]@l0@l0@C[2 1]@l0@l1@C[2 1]@l0@l0@C[2 1]@nt3@256C[2 1]@nnt123@void ifft_custom(input_cascade< cacc48, void > * sig_i, adf::output_buffer< cint32, adf::extents< 256 > > & restrict sig_o)t4@nonee[0 1]@e[0 1]@e[0 1]@e[0 1]@e[0 1]@nne[0 1]@e[0 1]@e[0 1]@e[0 1]@e[0 1]@e[0 1]@e[0 1]@e[0 1]@e[0 1]@  PortNames={'sig_i'; 'sig_o'}  PortSerializedTypes={'{P{Tinput_cascade{2{t{Scacc48}}{t{Bv}}}}}'; '{Q2{R{Tadf::output_buffer{2{t{Scint32}}{t{Tadf::extents{1{t{}256}}}}}}}}'}  PortWindowSizes={0.000000000000000000e+00, 2.560000000000000000e+02}  PortWindowMargins={0.000000000000000000e+00, 0.000000000000000000e+00}  PortSynchronicities={'auto', 'sync'}  PortSignalSizes={0.000000000000000000e+00; 0.000000000000000000e+00}  FunctionTemplateSpecKind=none  FunctionTemplateParamNames={}  FunctionTemplateParamKinds={}  FunctionTemplateParamTypes={}  FunctionTemplateParamValues={}  FunctionIndex=1  FunctionTabVisible=on  FunctionTemplateParamsVisible=off  FunctionDeclTypeOptions=C[1 1]@t124@void ifft_custom(input_cascade< cacc48, void > * sig_i, adf::output_buffer< cint32, adf::extents< 256 > > && restrict sig_o)  FunctionDecl=void ifft_custom(input_cascade< cacc48, void > * sig_i, adf::output_buffer< cint32, adf::extents< 256 > > && restrict sig_o)  FunctionTemplateParams={}  FunctionTemplateParamsEnables={}  PortAttrs={ 'input', 'sig_i', 'input_cascade< cacc48, void > *', '', '', '', ''; 'output', 'sig_o', 'adf::output_buffer< cint32, adf::extents< 256 > > & restrict', '256', '', 'sync', '' }  PortAttrsEnables={'off', 'off', 'off', 'off', 'off', 'off', 'off';'off', 'off', 'off', 'off', 'off', 'off', 'off'}  SampleTime=-1  KernelHeaderFile=customFFT_casc/ifft_custom.h  KernelFunction=ifft_custom  KernelInitFunction=ifft_custom_init  KernelSourceFile=customFFT_casc/ifft_custom.cpp  KernelSearchPaths={'./customFFT_casc'}  PreProcOptions={}  blockJsonConstraints="{\"type\":\"constraint\",\"constraintType\":\"stackSize\",\"sid\":\"5831\",\"lhs\":{\"type\":\"stackSize\",\"args\":{\"type\":\"kernel\",\"name\":\"OverlapSaveFIR_11paths/custom_11copies/ifft_custom7\",\"sid\":\"5831\"}},\"rhs\":{\"type\":\"value\",\"args\":{\"type\":\"evaluable\",\"expr\":\"4200\",\"value\":4200}},\"equality\":true}"
  ifft_custom8 : aieBasic/AIE Kernel  KernelAllAttrs=s[12;12;9;9;19;14;21;23;21;23;24;21;15;17;12;24;26;26;26;27;28;9;21;23;23;23;24;25;14;19;19;29]@FunctionNameDeclFileNamePortNamesPortTypesPortSerializedTypesPortDirectionsPortWindowSizeEnablesPortWindowMarginEnablesPortBufferSizeEnablesPortBufferMarginEnablesPortSynchronicityEnablesPortSignalSizeEnablesPortBufferSizesPortBufferMarginsFunctionDeclFunctionTemplateSpecKindFunctionTemplateParamNamesFunctionTemplateParamKindsFunctionTemplateParamTypesFunctionTemplateParamValuesFunctionTemplateParamEnablesClassDeclClassTemplateSpecKindClassTemplateParamNamesClassTemplateParamKindsClassTemplateParamTypesClassTemplateParamValuesClassTemplateParamEnablesClassCtorDeclsClassCtorParamNamesClassCtorParamTypesClassCtorParamSerializedTypes[1 1]@C[32 1]@t11@ifft_customt34@../../customFFT_casc/ifft_custom.hC[2 1]@t5@sig_it5@sig_oC[2 1]@t31@input_cascade< cacc48, void > *t60@adf::output_buffer< cint32, adf::extents< 256 > > & restrictC[2 1]@t41@{P{Tinput_cascade{2{t{Scacc48}}{t{Bv}}}}}t72@{Q2{R{Tadf::output_buffer{2{t{Scint32}}{t{Tadf::extents{1{t{}256}}}}}}}}C[2 1]@t5@inputt6@outputC[2 1]@l0@l1@C[2 1]@l0@l0@C[2 1]@l0@l1@C[2 1]@l0@l0@C[2 1]@l0@l1@C[2 1]@l0@l0@C[2 1]@nt3@256C[2 1]@nnt123@void ifft_custom(input_cascade< cacc48, void > * sig_i, adf::output_buffer< cint32, adf::extents< 256 > > & restrict sig_o)t4@nonee[0 1]@e[0 1]@e[0 1]@e[0 1]@e[0 1]@nne[0 1]@e[0 1]@e[0 1]@e[0 1]@e[0 1]@e[0 1]@e[0 1]@e[0 1]@e[0 1]@  PortNames={'sig_i'; 'sig_o'}  PortSerializedTypes={'{P{Tinput_cascade{2{t{Scacc48}}{t{Bv}}}}}'; '{Q2{R{Tadf::output_buffer{2{t{Scint32}}{t{Tadf::extents{1{t{}256}}}}}}}}'}  PortWindowSizes={0.000000000000000000e+00, 2.560000000000000000e+02}  PortWindowMargins={0.000000000000000000e+00, 0.000000000000000000e+00}  PortSynchronicities={'auto', 'sync'}  PortSignalSizes={0.000000000000000000e+00; 0.000000000000000000e+00}  FunctionTemplateSpecKind=none  FunctionTemplateParamNames={}  FunctionTemplateParamKinds={}  FunctionTemplateParamTypes={}  FunctionTemplateParamValues={}  FunctionIndex=1  FunctionTabVisible=on  FunctionTemplateParamsVisible=off  FunctionDeclTypeOptions=C[1 1]@t124@void ifft_custom(input_cascade< cacc48, void > * sig_i, adf::output_buffer< cint32, adf::extents< 256 > > && restrict sig_o)  FunctionDecl=void ifft_custom(input_cascade< cacc48, void > * sig_i, adf::output_buffer< cint32, adf::extents< 256 > > && restrict sig_o)  FunctionTemplateParams={}  FunctionTemplateParamsEnables={}  PortAttrs={ 'input', 'sig_i', 'input_cascade< cacc48, void > *', '', '', '', ''; 'output', 'sig_o', 'adf::output_buffer< cint32, adf::extents< 256 > > & restrict', '256', '', 'sync', '' }  PortAttrsEnables={'off', 'off', 'off', 'off', 'off', 'off', 'off';'off', 'off', 'off', 'off', 'off', 'off', 'off'}  SampleTime=-1  KernelHeaderFile=customFFT_casc/ifft_custom.h  KernelFunction=ifft_custom  KernelInitFunction=ifft_custom_init  KernelSourceFile=customFFT_casc/ifft_custom.cpp  KernelSearchPaths={'./customFFT_casc'}  PreProcOptions={}  blockJsonConstraints="{\"type\":\"constraint\",\"constraintType\":\"stackSize\",\"sid\":\"5832\",\"lhs\":{\"type\":\"stackSize\",\"args\":{\"type\":\"kernel\",\"name\":\"OverlapSaveFIR_11paths/custom_11copies/ifft_custom8\",\"sid\":\"5832\"}},\"rhs\":{\"type\":\"value\",\"args\":{\"type\":\"evaluable\",\"expr\":\"4200\",\"value\":4200}},\"equality\":true}"
  ifft_custom9 : aieBasic/AIE Kernel  KernelAllAttrs=s[12;12;9;9;19;14;21;23;21;23;24;21;15;17;12;24;26;26;26;27;28;9;21;23;23;23;24;25;14;19;19;29]@FunctionNameDeclFileNamePortNamesPortTypesPortSerializedTypesPortDirectionsPortWindowSizeEnablesPortWindowMarginEnablesPortBufferSizeEnablesPortBufferMarginEnablesPortSynchronicityEnablesPortSignalSizeEnablesPortBufferSizesPortBufferMarginsFunctionDeclFunctionTemplateSpecKindFunctionTemplateParamNamesFunctionTemplateParamKindsFunctionTemplateParamTypesFunctionTemplateParamValuesFunctionTemplateParamEnablesClassDeclClassTemplateSpecKindClassTemplateParamNamesClassTemplateParamKindsClassTemplateParamTypesClassTemplateParamValuesClassTemplateParamEnablesClassCtorDeclsClassCtorParamNamesClassCtorParamTypesClassCtorParamSerializedTypes[1 1]@C[32 1]@t11@ifft_customt34@../../customFFT_casc/ifft_custom.hC[2 1]@t5@sig_it5@sig_oC[2 1]@t31@input_cascade< cacc48, void > *t60@adf::output_buffer< cint32, adf::extents< 256 > > & restrictC[2 1]@t41@{P{Tinput_cascade{2{t{Scacc48}}{t{Bv}}}}}t72@{Q2{R{Tadf::output_buffer{2{t{Scint32}}{t{Tadf::extents{1{t{}256}}}}}}}}C[2 1]@t5@inputt6@outputC[2 1]@l0@l1@C[2 1]@l0@l0@C[2 1]@l0@l1@C[2 1]@l0@l0@C[2 1]@l0@l1@C[2 1]@l0@l0@C[2 1]@nt3@256C[2 1]@nnt123@void ifft_custom(input_cascade< cacc48, void > * sig_i, adf::output_buffer< cint32, adf::extents< 256 > > & restrict sig_o)t4@nonee[0 1]@e[0 1]@e[0 1]@e[0 1]@e[0 1]@nne[0 1]@e[0 1]@e[0 1]@e[0 1]@e[0 1]@e[0 1]@e[0 1]@e[0 1]@e[0 1]@  PortNames={'sig_i'; 'sig_o'}  PortSerializedTypes={'{P{Tinput_cascade{2{t{Scacc48}}{t{Bv}}}}}'; '{Q2{R{Tadf::output_buffer{2{t{Scint32}}{t{Tadf::extents{1{t{}256}}}}}}}}'}  PortWindowSizes={0.000000000000000000e+00, 2.560000000000000000e+02}  PortWindowMargins={0.000000000000000000e+00, 0.000000000000000000e+00}  PortSynchronicities={'auto', 'sync'}  PortSignalSizes={0.000000000000000000e+00; 0.000000000000000000e+00}  FunctionTemplateSpecKind=none  FunctionTemplateParamNames={}  FunctionTemplateParamKinds={}  FunctionTemplateParamTypes={}  FunctionTemplateParamValues={}  FunctionIndex=1  FunctionTabVisible=on  FunctionTemplateParamsVisible=off  FunctionDeclTypeOptions=C[1 1]@t124@void ifft_custom(input_cascade< cacc48, void > * sig_i, adf::output_buffer< cint32, adf::extents< 256 > > && restrict sig_o)  FunctionDecl=void ifft_custom(input_cascade< cacc48, void > * sig_i, adf::output_buffer< cint32, adf::extents< 256 > > && restrict sig_o)  FunctionTemplateParams={}  FunctionTemplateParamsEnables={}  PortAttrs={ 'input', 'sig_i', 'input_cascade< cacc48, void > *', '', '', '', ''; 'output', 'sig_o', 'adf::output_buffer< cint32, adf::extents< 256 > > & restrict', '256', '', 'sync', '' }  PortAttrsEnables={'off', 'off', 'off', 'off', 'off', 'off', 'off';'off', 'off', 'off', 'off', 'off', 'off', 'off'}  SampleTime=-1  KernelHeaderFile=customFFT_casc/ifft_custom.h  KernelFunction=ifft_custom  KernelInitFunction=ifft_custom_init  KernelSourceFile=customFFT_casc/ifft_custom.cpp  KernelSearchPaths={'./customFFT_casc'}  PreProcOptions={}  blockJsonConstraints="{\"type\":\"constraint\",\"constraintType\":\"stackSize\",\"sid\":\"5833\",\"lhs\":{\"type\":\"stackSize\",\"args\":{\"type\":\"kernel\",\"name\":\"OverlapSaveFIR_11paths/custom_11copies/ifft_custom9\",\"sid\":\"5833\"}},\"rhs\":{\"type\":\"value\",\"args\":{\"type\":\"evaluable\",\"expr\":\"4200\",\"value\":4200}},\"equality\":true}"
  Out1 : Outport
  Out2 : Outport  Port=2
  Out3 : Outport  Port=3
  Out4 : Outport  Port=4
  Out5 : Outport  Port=5
  Out6 : Outport  Port=6
  Out7 : Outport  Port=7
  Out8 : Outport  Port=8
  Out9 : Outport  Port=9
  Out10 : Outport  Port=10
  Out11 : Outport  Port=11
  wires:
  PLIO/1 -> fft_custom/1
  In1/1 -> PLIO/1
  ifft_custom/1 -> PLIO1/1
  PLIO1/1 -> Out1/1
  PLIO2/1 -> fft_custom1/1
  In2/1 -> PLIO2/1
  ifft_custom1/1 -> PLIO3/1
  PLIO3/1 -> Out2/1
  PLIO6/1 -> fft_custom3/1
  PLIO5/1 -> Out3/1
  PLIO7/1 -> Out4/1
  In4/1 -> PLIO6/1
  In3/1 -> PLIO4/1
  ifft_custom3/1 -> PLIO7/1
  ifft_custom2/1 -> PLIO5/1
  PLIO4/1 -> fft_custom2/1
  ifft_custom6/1 -> PLIO13/1
  PLIO8/1 -> fft_custom4/1
  PLIO13/1 -> Out7/1
  In5/1 -> PLIO8/1
  PLIO9/1 -> Out5/1
  In7/1 -> PLIO12/1
  PLIO11/1 -> Out6/1
  ifft_custom5/1 -> PLIO11/1
  PLIO12/1 -> fft_custom6/1
  In6/1 -> PLIO10/1
  PLIO10/1 -> fft_custom5/1
  ifft_custom4/1 -> PLIO9/1
  fft_custom/1 -> ifft_custom/1
  fft_custom1/1 -> ifft_custom1/1
  fft_custom3/1 -> ifft_custom3/1
  fft_custom2/1 -> ifft_custom2/1
  fft_custom5/1 -> ifft_custom5/1
  fft_custom6/1 -> ifft_custom6/1
  fft_custom4/1 -> ifft_custom4/1
  In8/1 -> PLIO18/1
  PLIO21/1 -> Out9/1
  ifft_custom10/1 -> PLIO17/1
  PLIO17/1 -> Out11/1
  ifft_custom7/1 -> PLIO19/1
  ifft_custom9/1 -> PLIO15/1
  PLIO14/1 -> fft_custom9/1
  In9/1 -> PLIO20/1
  PLIO16/1 -> fft_custom10/1
  fft_custom9/1 -> ifft_custom9/1
  PLIO20/1 -> fft_custom8/1
  fft_custom8/1 -> ifft_custom8/1
  PLIO19/1 -> Out8/1
  ifft_custom8/1 -> PLIO21/1
  fft_custom10/1 -> ifft_custom10/1
  PLIO18/1 -> fft_custom7/1
  fft_custom7/1 -> ifft_custom7/1
  In11/1 -> PLIO16/1
  PLIO15/1 -> Out10/1
  In10/1 -> PLIO14/1
